simulink model "deltino"  (R2021b)
(part 9 of 10)

et152 = t27.*th33_dot.*(-1.6125e-2)+t28.*th41_dot.*(3.0./2.5e+2)-t29.*th42_dot.*1.6125e-2-t30.*th43_dot.*1.6125e-2-(t75.*th11_dot)./3.75e+2-(t76.*th12_dot)./1.5e+3-(t77.*th13_dot)./1.5e+3-(t78.*th21_dot)./3.75e+2-(t79.*th22_dot)./1.5e+3-(t80.*th23_dot)./1.5e+3-(t81.*th31_dot)./3.75e+2-(t82.*th32_dot)./1.5e+3-(t83.*th33_dot)./1.5e+3-(t84.*th41_dot)./3.75e+2-(t85.*th42_dot)./1.5e+3-(t86.*th43_dot)./1.5e+3-psi_dot.*t19.*t46.*(2.1e+1./1.0e+3)-psi_dot.*t20.*t46.*(2.1e+1./1.0e+3)-psi_dot.*t21.*t46.*(2.1e+1./1.0e+3);
et153 = psi_dot.*t22.*t46.*(2.1e+1./1.0e+3)+psi_dot.*t23.*t46.*(2.1e+1./1.0e+3)+psi_dot.*t24.*t46.*(2.1e+1./1.0e+3)+psi_dot.*t25.*t46.*(2.1e+1./1.0e+3)+psi_dot.*t26.*t46.*(2.1e+1./1.0e+3)+psi_dot.*t27.*t46.*(2.1e+1./1.0e+3)-psi_dot.*t28.*t46.*(2.1e+1./1.0e+3)-psi_dot.*t29.*t46.*(2.1e+1./1.0e+3)-psi_dot.*t30.*t46.*(2.1e+1./1.0e+3)+psi_dot.*t5.*t74.*6.75e-3+psi_dot.*t6.*t74.*6.75e-3+psi_dot.*t8.*t74.*6.75e-3+psi_dot.*t9.*t74.*6.75e-3+psi_dot.*t11.*t74.*6.75e-3+psi_dot.*t12.*t74.*6.75e-3+psi_dot.*t14.*t74.*6.75e-3+psi_dot.*t15.*t74.*6.75e-3-psi_dot.*t19.*t74.*(3.0./5.0e+2);
et154 = psi_dot.*t20.*t74.*(-3.0./5.0e+2)-psi_dot.*t21.*t74.*(3.0./5.0e+2)-psi_dot.*t22.*t74.*(3.0./5.0e+2)-psi_dot.*t23.*t74.*(3.0./5.0e+2)-psi_dot.*t24.*t74.*(3.0./5.0e+2)-psi_dot.*t25.*t74.*(3.0./5.0e+2)-psi_dot.*t26.*t74.*(3.0./5.0e+2)-psi_dot.*t27.*t74.*(3.0./5.0e+2)-psi_dot.*t28.*t74.*(3.0./5.0e+2)-psi_dot.*t29.*t74.*(3.0./5.0e+2)-psi_dot.*t30.*t74.*(3.0./5.0e+2)+(psi_dot.*t48.*t74)./3.75e+2+psi_dot.*t49.*t74.*4.666666666666667e-3+psi_dot.*t50.*t74.*4.666666666666667e-3+(psi_dot.*t51.*t74)./3.75e+2+psi_dot.*t52.*t74.*4.666666666666667e-3+psi_dot.*t53.*t74.*4.666666666666667e-3+(psi_dot.*t54.*t74)./3.75e+2+psi_dot.*t55.*t74.*4.666666666666667e-3+psi_dot.*t56.*t74.*4.666666666666667e-3;
et155 = (psi_dot.*t57.*t74)./3.75e+2+psi_dot.*t58.*t74.*4.666666666666667e-3+psi_dot.*t59.*t74.*4.666666666666667e-3+t4.*t46.*th11_dot.*(3.0./1.0e+3)+t5.*t46.*th12_dot.*(3.0./1.0e+3)+t6.*t46.*th13_dot.*(3.0./1.0e+3)+t7.*t46.*th21_dot.*(3.0./1.0e+3)+t8.*t46.*th22_dot.*(3.0./1.0e+3)+t9.*t46.*th23_dot.*(3.0./1.0e+3)+t20.*t46.*th12_dot.*3.375e-3+t21.*t46.*th13_dot.*3.375e-3+t10.*t46.*th31_dot.*(3.0./1.0e+3)-t4.*t74.*th11_dot.*1.05e-2+t11.*t46.*th32_dot.*(3.0./1.0e+3)-t5.*t74.*th12_dot.*1.05e-2+t12.*t46.*th33_dot.*(3.0./1.0e+3)+t23.*t46.*th22_dot.*3.375e-3-t6.*t74.*th13_dot.*1.05e-2+t24.*t46.*th23_dot.*3.375e-3;
et156 = t13.*t46.*th41_dot.*(3.0./1.0e+3)+t7.*t74.*th21_dot.*1.05e-2+t14.*t46.*th42_dot.*(3.0./1.0e+3)+t8.*t74.*th22_dot.*1.05e-2+t15.*t46.*th43_dot.*(3.0./1.0e+3)+t26.*t46.*th32_dot.*3.375e-3+t9.*t74.*th23_dot.*1.05e-2+t27.*t46.*th33_dot.*3.375e-3+t10.*t74.*th31_dot.*1.05e-2+t11.*t74.*th32_dot.*1.05e-2+t29.*t46.*th42_dot.*3.375e-3+t12.*t74.*th33_dot.*1.05e-2+t30.*t46.*th43_dot.*3.375e-3-t20.*t92.*th12_dot.*5.25e-3+t21.*t92.*th13_dot.*5.25e-3-t13.*t74.*th41_dot.*1.05e-2-t14.*t74.*th42_dot.*1.05e-2-t15.*t74.*th43_dot.*1.05e-2;
et157 = (t46.*t75.*th11_dot)./3.75e+2+t46.*t76.*th12_dot.*4.666666666666667e-3+t46.*t77.*th13_dot.*4.666666666666667e-3+t23.*t92.*th22_dot.*5.25e-3-t24.*t92.*th23_dot.*5.25e-3+(t46.*t78.*th21_dot)./3.75e+2+t46.*t79.*th22_dot.*4.666666666666667e-3+t46.*t80.*th23_dot.*4.666666666666667e-3+t26.*t92.*th32_dot.*5.25e-3-t27.*t92.*th33_dot.*5.25e-3+(t46.*t81.*th31_dot)./3.75e+2+t46.*t82.*th32_dot.*4.666666666666667e-3+t46.*t83.*th33_dot.*4.666666666666667e-3-t29.*t92.*th42_dot.*5.25e-3+t30.*t92.*th43_dot.*5.25e-3+(t46.*t84.*th41_dot)./3.75e+2+t46.*t85.*th42_dot.*4.666666666666667e-3+t46.*t86.*th43_dot.*4.666666666666667e-3-psi_dot.*t5.*t46.*t92.*(3.0./1.0e+3);
et158 = psi_dot.*t6.*t46.*t92.*(3.0./1.0e+3)-psi_dot.*t8.*t46.*t92.*(3.0./1.0e+3)+psi_dot.*t9.*t46.*t92.*(3.0./1.0e+3)-psi_dot.*t11.*t46.*t92.*(3.0./1.0e+3)+psi_dot.*t12.*t46.*t92.*(3.0./1.0e+3)-psi_dot.*t14.*t46.*t92.*(3.0./1.0e+3)+psi_dot.*t15.*t46.*t92.*(3.0./1.0e+3)-psi_dot.*t20.*t46.*t92.*4.5e-3+psi_dot.*t21.*t46.*t92.*4.5e-3-psi_dot.*t23.*t46.*t92.*4.5e-3+psi_dot.*t24.*t46.*t92.*4.5e-3-psi_dot.*t26.*t46.*t92.*4.5e-3+psi_dot.*t27.*t46.*t92.*4.5e-3-psi_dot.*t29.*t46.*t92.*4.5e-3+psi_dot.*t30.*t46.*t92.*4.5e-3+psi_dot.*t5.*t74.*t92.*1.05e-2;
et159 = psi_dot.*t6.*t74.*t92.*(-1.05e-2)-psi_dot.*t8.*t74.*t92.*1.05e-2+psi_dot.*t9.*t74.*t92.*1.05e-2-psi_dot.*t11.*t74.*t92.*1.05e-2+psi_dot.*t12.*t74.*t92.*1.05e-2+psi_dot.*t14.*t74.*t92.*1.05e-2-psi_dot.*t15.*t74.*t92.*1.05e-2-(psi_dot.*t46.*t76.*t92)./3.75e+2+(psi_dot.*t46.*t77.*t92)./3.75e+2-(psi_dot.*t46.*t79.*t92)./3.75e+2+(psi_dot.*t46.*t80.*t92)./3.75e+2-(psi_dot.*t46.*t82.*t92)./3.75e+2+(psi_dot.*t46.*t83.*t92)./3.75e+2-(psi_dot.*t46.*t85.*t92)./3.75e+2+(psi_dot.*t46.*t86.*t92)./3.75e+2+t20.*t46.*t92.*th12_dot.*5.25e-3-t21.*t46.*t92.*th13_dot.*5.25e-3;
et160 = t5.*t74.*t92.*th12_dot.*(-2.25e-3)-t23.*t46.*t92.*th22_dot.*5.25e-3+t6.*t74.*t92.*th13_dot.*2.25e-3+t24.*t46.*t92.*th23_dot.*5.25e-3-t8.*t74.*t92.*th22_dot.*2.25e-3-t26.*t46.*t92.*th32_dot.*5.25e-3+t9.*t74.*t92.*th23_dot.*2.25e-3+t20.*t74.*t92.*th12_dot.*1.5e-3+t27.*t46.*t92.*th33_dot.*5.25e-3-t21.*t74.*t92.*th13_dot.*1.5e-3-t11.*t74.*t92.*th32_dot.*2.25e-3+t29.*t46.*t92.*th42_dot.*5.25e-3+t12.*t74.*t92.*th33_dot.*2.25e-3+t23.*t74.*t92.*th22_dot.*1.5e-3-t30.*t46.*t92.*th43_dot.*5.25e-3-t24.*t74.*t92.*th23_dot.*1.5e-3;
et161 = t14.*t74.*t92.*th42_dot.*(-2.25e-3)+t15.*t74.*t92.*th43_dot.*2.25e-3+t26.*t74.*t92.*th32_dot.*1.5e-3-t27.*t74.*t92.*th33_dot.*1.5e-3-(t49.*t74.*t92.*th12_dot)./3.75e+2+(t50.*t74.*t92.*th13_dot)./3.75e+2+t29.*t74.*t92.*th42_dot.*1.5e-3-t30.*t74.*t92.*th43_dot.*1.5e-3-(t52.*t74.*t92.*th22_dot)./3.75e+2+(t53.*t74.*t92.*th23_dot)./3.75e+2-(t55.*t74.*t92.*th32_dot)./3.75e+2+(t56.*t74.*t92.*th33_dot)./3.75e+2-(t58.*t74.*t92.*th42_dot)./3.75e+2+(t59.*t74.*t92.*th43_dot)./3.75e+2;
et162 = -t138+t139+t140-t141+t142+t143-t144+t145+t146-t147+t148+t149+t189+t191+t193+t195+t197+t199+t201+t203+t205+t207+t209+t211-t329-t330-t331-t332-t333-t334-t335-t336-t337-t338-t339-t340+t341+t343+t345+t347+t351+t353-t355-t357+t406+t407+t408+t409+t410+t411+t412+t413-t470-t471-t472-t473+t503+t504+t506+t507+t509+t510+t512+t513-t567-t569-t571-t573-t575-t577-t579-t581+t598-t600-t601-t602-t603-t604-t605-t606-t607+t616+t617+t618+t619+t653;
et163 = t654+t655+t656-t683+t685+t687-t689+t691+t693-t695-t697+t699+t701-t703-t705+t707+t709+t711+t713-t715-t717-t719-t721+t769+t770+t771+t772+t773+t774+t775+t776+t777+t778+t779+t780+t829-t830-t831+t832-t833-t834+t835-t836-t837+t838-t839-t840-t889-t890-t891+t892+t893+t894+t895+t896+t897-t898-t899-t900+t901+t902+t903+t904+t905+t906+t907+t908+t934+t951+t952+t953+t954+t955+t956+t957+t958-t1275-t1276-t1277+t1278+t1279+t1280+t1281+t1282+t1283-t1284-t1285-t1286-t1340-t1341-t1342-t1343-t1344;
et164 = -t1345-t1346-t1347+t1444-t1445+t1446-t1447+t1449+t1451-t1458+t1464-t1465-t1468+t1469-t1472+t1473+t1474-t1475-t1549+t1550-t1551+t1552-t1553+t1554-t1555+t1556+t1571+t1573+t1575+t1577+t1646+t1647+t1648+t1649-t1675+t1676-t1677+t1678+t1679-t1680-t1681+t1682-t1683+t1684-t1685+t1686-t1687+t1688+t1689-t1690-t1751+t1752-t1753+t1754-t1755+t1756-t1757+t1758-t1808+t1809-t1810+t1811-t1812+t1813-t1814+t1815+t1849-t1850+t1851-t1852+t1853-t1854+t1855-t1856+t1878+t1879+t1881+t1884-t1933+t1934-t1935+t1936-t1937+t1938-t1939+t1940;
et165 = -t2002+t2003-t2004+t2005-t2006+t2007-t2008+t2009-psi_dot.*t3.*t4.*(3.0./5.0e+2)+psi_dot.*t3.*t5.*(3.0./1.0e+3)+psi_dot.*t3.*t6.*(3.0./1.0e+3)-psi_dot.*t3.*t7.*(3.0./5.0e+2)+psi_dot.*t3.*t8.*(3.0./1.0e+3)+psi_dot.*t3.*t9.*(3.0./1.0e+3)-psi_dot.*t3.*t10.*(3.0./5.0e+2)+psi_dot.*t3.*t11.*(3.0./1.0e+3)+psi_dot.*t3.*t12.*(3.0./1.0e+3)-psi_dot.*t3.*t13.*(3.0./5.0e+2)+psi_dot.*t3.*t14.*(3.0./1.0e+3)+psi_dot.*t3.*t15.*(3.0./1.0e+3)-psi_dot.*t3.*t19.*(3.0./1.0e+2)+psi_dot.*t4.*t18.*(2.1e+1./1.0e+3)-psi_dot.*t3.*t20.*1.65e-2-psi_dot.*t5.*t18.*1.05e-2-psi_dot.*t3.*t21.*1.65e-2;
et166 = psi_dot.*t6.*t18.*(-1.05e-2)-psi_dot.*t3.*t22.*(3.0./1.0e+2)-psi_dot.*t7.*t18.*(2.1e+1./1.0e+3)-psi_dot.*t3.*t23.*1.65e-2+psi_dot.*t8.*t18.*1.05e-2-psi_dot.*t3.*t24.*1.65e-2+psi_dot.*t9.*t18.*1.05e-2+psi_dot.*t3.*t25.*(3.0./2.5e+2)-psi_dot.*t10.*t18.*(2.1e+1./1.0e+3)+psi_dot.*t3.*t26.*2.55e-2+psi_dot.*t11.*t18.*1.05e-2+psi_dot.*t3.*t27.*2.55e-2+psi_dot.*t12.*t18.*1.05e-2+psi_dot.*t3.*t28.*(3.0./2.5e+2)+psi_dot.*t13.*t18.*(2.1e+1./1.0e+3)+psi_dot.*t3.*t29.*2.55e-2-psi_dot.*t14.*t18.*1.05e-2+psi_dot.*t3.*t30.*2.55e-2;
et167 = psi_dot.*t15.*t18.*(-1.05e-2)-psi_dot.*t3.*t75.*(2.0./3.75e+2)+(psi_dot.*t3.*t76)./3.75e+2+(psi_dot.*t3.*t77)./3.75e+2-psi_dot.*t3.*t78.*(2.0./3.75e+2)+(psi_dot.*t3.*t79)./3.75e+2+(psi_dot.*t3.*t80)./3.75e+2-psi_dot.*t3.*t81.*(2.0./3.75e+2)+(psi_dot.*t3.*t82)./3.75e+2+(psi_dot.*t3.*t83)./3.75e+2-psi_dot.*t3.*t84.*(2.0./3.75e+2)+(psi_dot.*t3.*t85)./3.75e+2+(psi_dot.*t3.*t86)./3.75e+2+t18.*t92.*t125+t18.*t92.*t128-t4.*t18.*th11_dot.*(3.0./1.0e+2)-t5.*t18.*th12_dot.*1.65e-2-t6.*t18.*th13_dot.*1.65e-2-t7.*t18.*th21_dot.*(3.0./1.0e+2)-t8.*t18.*th22_dot.*1.65e-2-t9.*t18.*th23_dot.*1.65e-2;
et168 = t10.*t18.*th31_dot.*(3.0./2.5e+2)+t11.*t18.*th32_dot.*2.55e-2+t12.*t18.*th33_dot.*2.55e-2+t13.*t18.*th41_dot.*(3.0./2.5e+2)+t14.*t18.*th42_dot.*2.55e-2+t15.*t18.*th43_dot.*2.55e-2-phi_dot.*t5.*t16.*t46.*6.75e-3-phi_dot.*t6.*t16.*t46.*6.75e-3-phi_dot.*t8.*t16.*t46.*6.75e-3-phi_dot.*t9.*t16.*t46.*6.75e-3-phi_dot.*t11.*t16.*t46.*6.75e-3-phi_dot.*t12.*t16.*t46.*6.75e-3-phi_dot.*t14.*t16.*t46.*6.75e-3-phi_dot.*t15.*t16.*t46.*6.75e-3-(phi_dot.*t16.*t46.*t48)./3.75e+2-(phi_dot.*t16.*t46.*t51)./3.75e+2-(phi_dot.*t16.*t46.*t54)./3.75e+2;
et169 = phi_dot.*t16.*t46.*t57.*(-1.0./3.75e+2)-psi_dot.*t6.*t18.*t92.*(3.0./5.0e+2)-psi_dot.*t9.*t18.*t92.*(3.0./5.0e+2)-psi_dot.*t11.*t18.*t92.*(3.0./2.0e+2)+psi_dot.*t12.*t18.*t92.*(3.0./2.0e+2)-psi_dot.*t14.*t18.*t92.*(3.0./2.0e+2)+psi_dot.*t15.*t18.*t92.*(3.0./2.0e+2)-(psi_dot.*t18.*t49.*t92)./7.5e+2+(psi_dot.*t18.*t50.*t92)./7.5e+2-(psi_dot.*t18.*t52.*t92)./7.5e+2+(psi_dot.*t18.*t53.*t92)./7.5e+2-(psi_dot.*t18.*t55.*t92)./7.5e+2+(psi_dot.*t18.*t56.*t92)./7.5e+2-(psi_dot.*t18.*t58.*t92)./7.5e+2+(psi_dot.*t18.*t59.*t92)./7.5e+2+t3.*t20.*t92.*th12_dot.*8.25e-3-t3.*t21.*t92.*th13_dot.*8.25e-3;
et170 = t3.*t23.*t92.*th22_dot.*8.25e-3-t3.*t24.*t92.*th23_dot.*8.25e-3-t3.*t26.*t92.*th32_dot.*1.275e-2+t3.*t27.*t92.*th33_dot.*1.275e-2-t3.*t29.*t92.*th42_dot.*1.275e-2+t3.*t30.*t92.*th43_dot.*1.275e-2-phi_dot.*t5.*t18.*t31.*t92.*(3.0./5.0e+2)-phi_dot.*t8.*t18.*t31.*t92.*(3.0./5.0e+2)-phi_dot.*t5.*t16.*t46.*t92.*1.05e-2-phi_dot.*t9.*t16.*t46.*t92.*1.05e-2-phi_dot.*t12.*t16.*t46.*t92.*1.05e-2-phi_dot.*t14.*t16.*t46.*t92.*1.05e-2;
et171 = t304+t305+t306+t307+t308+t309+t310+t311+t312+t313+t314+t315+t462+t463+t464+t465+t466+t467+t468+t469+t586+t587+t588+t589+t590+t591+t592+t593+t594+t595+t596+t597-t667-t668+t669+t670+t753+t756+t759+t762-t817-t818-t819-t820-t821-t822-t824-t825-t827-t828+t877+t878+t879-t880-t881-t882-t883-t884-t885+t886+t887+t888+t961+t963+t965+t967+t969+t971+t973+t975+t976+t977+t978-t979-t980-t981-t982-t983-t984+t985+t986+t987+t1002+t1003+t1004+t1005+t1006+t1007+t1008+t1009+t1054+t1055+t1056+t1057+t1058+t1059+t1060+t1061+t1062+t1063+t1064+t1065-t1106+t1107+t1108-t1109+t1110+t1111-t1112+t1113+t1114-t1115+t1116+t1117+t1119+t1120;
et172 = t1122+t1123-t1124-t1125-t1128-t1129+t1132+t1133-t1162-t1163-t1166-t1167+t1170+t1171+t1172+t1173-t1183-t1184-t1185-t1186-t1187-t1188-t1190-t1191-t1193-t1194+t1247+t1248+t1249+t1250+t1251+t1252+t1253+t1254+t1307+t1332+t1335+t1337+t1338-t1360-t1361-t1362+t1363+t1364+t1365+t1366+t1367+t1368-t1369-t1370-t1371+t1512+t1513+t1514+t1515+t1541-t1542+t1543-t1544+t1545-t1546+t1547-t1548+t1590+t1591+t1592+t1593+t1594+t1595+t1596+t1597+t1598+t1608+t1609+t1610+t1611+t1612+t1613+t1614+t1615+t1616+t1617+t1618+t1619+t1637+t1639+t1641+t1643+t1659-t1660+t1661-t1662+t1665-t1666+t1669-t1670+t1711-t1712+t1713;
et173 = -t1714+t1716+t1718+t1719+t1721+t1723+t1725+t1760+t1762+t1764+t1766+t1865+t1866+t1867+t1868+t1869-t1870+t1871-t1872+t1873-t1874+t1875-t1876+t1909+t1912+t1914+t1915+t1971+t1973+t1975+t1977+t1994-t1995+t1996-t1997+t1998-t1999+t2000-t2001+t2034-t2035+t2036-t2037+t2038-t2039+t2040-t2041-t2108+t2109-t2110+t2111-t2112+t2113-t2114+t2115-t2124+t2125-t2126+t2127-t2128+t2129-t2130+t2131+t2150+t2153+t2155+t2156-t16.*zeta_dot.*6.720125e-1+t3.*t31.*t153+t3.*t31.*t154-t3.*t16.*th11_dot.*(4.0./3.75e+2)+t3.*t16.*th12_dot.*(2.0./3.75e+2)+t3.*t16.*th13_dot.*(2.0./3.75e+2)-t3.*t16.*th21_dot.*(4.0./3.75e+2);
et174 = t3.*t16.*th22_dot.*(2.0./3.75e+2)+t3.*t16.*th23_dot.*(2.0./3.75e+2)-t3.*t16.*th31_dot.*(4.0./3.75e+2)+t3.*t16.*th32_dot.*(2.0./3.75e+2)+t3.*t16.*th33_dot.*(2.0./3.75e+2)-t3.*t16.*th41_dot.*(4.0./3.75e+2)+t3.*t16.*th42_dot.*(2.0./3.75e+2)+t3.*t16.*th43_dot.*(2.0./3.75e+2)-t5.*t16.*zeta_dot.*1.35e-2-t6.*t16.*zeta_dot.*1.35e-2-t8.*t16.*zeta_dot.*1.35e-2-t9.*t16.*zeta_dot.*1.35e-2-t11.*t16.*zeta_dot.*1.35e-2-t12.*t16.*zeta_dot.*1.35e-2-t14.*t16.*zeta_dot.*1.35e-2-t15.*t16.*zeta_dot.*1.35e-2-(t16.*t61.*zeta_dot)./1.25e+2-(t16.*t62.*zeta_dot)./1.25e+2-(t16.*t64.*zeta_dot)./1.25e+2;
et175 = t16.*t65.*zeta_dot.*(-1.0./1.25e+2)-(t16.*t67.*zeta_dot)./1.25e+2-(t16.*t68.*zeta_dot)./1.25e+2-(t16.*t70.*zeta_dot)./1.25e+2-(t16.*t71.*zeta_dot)./1.25e+2-t3.*t16.*t19.*th11_dot.*(3.0./5.0e+2)+t3.*t16.*t20.*th12_dot.*(3.0./1.0e+3)+t3.*t16.*t21.*th13_dot.*(3.0./1.0e+3)-t3.*t16.*t22.*th21_dot.*(3.0./5.0e+2)+t3.*t16.*t23.*th22_dot.*(3.0./1.0e+3)+t16.*t18.*t19.*th11_dot.*(2.1e+1./1.0e+3)+t3.*t16.*t24.*th23_dot.*(3.0./1.0e+3)-t16.*t18.*t20.*th12_dot.*1.05e-2-t16.*t18.*t21.*th13_dot.*1.05e-2-t3.*t16.*t25.*th31_dot.*(3.0./5.0e+2)+t3.*t16.*t26.*th32_dot.*(3.0./1.0e+3)-t16.*t18.*t22.*th21_dot.*(2.1e+1./1.0e+3)+t3.*t16.*t27.*th33_dot.*(3.0./1.0e+3);
et176 = t16.*t18.*t23.*th22_dot.*1.05e-2+t16.*t18.*t24.*th23_dot.*1.05e-2-t3.*t16.*t28.*th41_dot.*(3.0./5.0e+2)+t3.*t16.*t29.*th42_dot.*(3.0./1.0e+3)-t16.*t18.*t25.*th31_dot.*(2.1e+1./1.0e+3)+t3.*t16.*t30.*th43_dot.*(3.0./1.0e+3)+t16.*t18.*t26.*th32_dot.*1.05e-2+t16.*t18.*t27.*th33_dot.*1.05e-2+t16.*t18.*t28.*th41_dot.*(2.1e+1./1.0e+3)-t16.*t18.*t29.*th42_dot.*1.05e-2-t16.*t18.*t30.*th43_dot.*1.05e-2-t3.*t4.*t31.*zeta_dot.*(3.0./5.0e+2)+t3.*t5.*t31.*zeta_dot.*(3.0./1.0e+3)+t3.*t6.*t31.*zeta_dot.*(3.0./1.0e+3)-t3.*t7.*t31.*zeta_dot.*(3.0./5.0e+2)+t3.*t8.*t31.*zeta_dot.*(3.0./1.0e+3)+t3.*t9.*t31.*zeta_dot.*(3.0./1.0e+3);
et177 = t3.*t10.*t31.*zeta_dot.*(-3.0./5.0e+2)+t3.*t11.*t31.*zeta_dot.*(3.0./1.0e+3)+t3.*t12.*t31.*zeta_dot.*(3.0./1.0e+3)-t3.*t13.*t31.*zeta_dot.*(3.0./5.0e+2)+t3.*t14.*t31.*zeta_dot.*(3.0./1.0e+3)+t3.*t15.*t31.*zeta_dot.*(3.0./1.0e+3)-t3.*t19.*t31.*zeta_dot.*(3.0./1.0e+2)+t4.*t18.*t31.*zeta_dot.*(2.1e+1./1.0e+3)-t3.*t20.*t31.*zeta_dot.*1.65e-2-t5.*t18.*t31.*zeta_dot.*1.05e-2-t3.*t21.*t31.*zeta_dot.*1.65e-2-t6.*t18.*t31.*zeta_dot.*1.05e-2-t3.*t22.*t31.*zeta_dot.*(3.0./1.0e+2)-t7.*t18.*t31.*zeta_dot.*(2.1e+1./1.0e+3)-t3.*t23.*t31.*zeta_dot.*1.65e-2+t8.*t18.*t31.*zeta_dot.*1.05e-2;
et178 = t3.*t24.*t31.*zeta_dot.*(-1.65e-2)+t9.*t18.*t31.*zeta_dot.*1.05e-2-t10.*t18.*t31.*zeta_dot.*(2.1e+1./1.0e+3)+t3.*t26.*t31.*zeta_dot.*2.55e-2+t11.*t18.*t31.*zeta_dot.*1.05e-2+t3.*t27.*t31.*zeta_dot.*2.55e-2+t12.*t18.*t31.*zeta_dot.*1.05e-2+t13.*t18.*t31.*zeta_dot.*(2.1e+1./1.0e+3)+t3.*t29.*t31.*zeta_dot.*2.55e-2-t14.*t18.*t31.*zeta_dot.*1.05e-2+t3.*t30.*t31.*zeta_dot.*2.55e-2-t15.*t18.*t31.*zeta_dot.*1.05e-2-t16.*t25.*t47.*zeta_dot.*(3.0./2.5e+2)-t16.*t28.*t47.*zeta_dot.*(3.0./2.5e+2)-t5.*t16.*t92.*zeta_dot.*(2.1e+1./1.0e+3)+t6.*t16.*t92.*zeta_dot.*(2.1e+1./1.0e+3);
et179 = t8.*t16.*t92.*zeta_dot.*(2.1e+1./1.0e+3)-t9.*t16.*t92.*zeta_dot.*(2.1e+1./1.0e+3)+t11.*t16.*t92.*zeta_dot.*(2.1e+1./1.0e+3)-t12.*t16.*t92.*zeta_dot.*(2.1e+1./1.0e+3)-t14.*t16.*t92.*zeta_dot.*(2.1e+1./1.0e+3)+t15.*t16.*t92.*zeta_dot.*(2.1e+1./1.0e+3)-phi_dot.*t3.*t4.*t16.*t31.*(2.1e+1./1.0e+3)-phi_dot.*t3.*t13.*t16.*t31.*(2.1e+1./1.0e+3)-phi_dot.*t4.*t16.*t18.*t31.*(3.0./5.0e+2)-phi_dot.*t7.*t16.*t18.*t31.*(3.0./5.0e+2)-phi_dot.*t10.*t16.*t18.*t31.*(3.0./5.0e+2)-phi_dot.*t13.*t16.*t18.*t31.*(3.0./5.0e+2)-phi_dot.*t3.*t18.*t25.*t73.*(3.0./2.5e+2)-phi_dot.*t3.*t18.*t28.*t73.*(3.0./2.5e+2)-phi_dot.*t6.*t21.*t73.*t92.*(2.0./3.75e+2)-phi_dot.*t9.*t24.*t73.*t92.*(2.0./3.75e+2);
et180 = phi_dot.*t12.*t27.*t73.*t92.*(-2.0./3.75e+2)-phi_dot.*t15.*t30.*t73.*t92.*(2.0./3.75e+2)-phi_dot.*t5.*t47.*t73.*t92.*(3.0./5.0e+2)-phi_dot.*t8.*t47.*t73.*t92.*(3.0./5.0e+2)-phi_dot.*t11.*t47.*t73.*t92.*(3.0./5.0e+2)-phi_dot.*t14.*t47.*t73.*t92.*(3.0./5.0e+2)-t16.*t18.*t20.*t92.*th12_dot.*2.25e-3+t16.*t18.*t21.*t92.*th13_dot.*2.25e-3-t16.*t18.*t23.*t92.*th22_dot.*2.25e-3+t16.*t18.*t24.*t92.*th23_dot.*2.25e-3-t16.*t18.*t26.*t92.*th32_dot.*2.25e-3+t16.*t18.*t27.*t92.*th33_dot.*2.25e-3-t16.*t18.*t29.*t92.*th42_dot.*2.25e-3+t16.*t18.*t30.*t92.*th43_dot.*2.25e-3-t3.*t4.*t19.*t31.*zeta_dot.*(4.0./3.75e+2);
et181 = t3.*t5.*t20.*t31.*zeta_dot.*(2.0./3.75e+2)+t3.*t6.*t21.*t31.*zeta_dot.*(2.0./3.75e+2)-t3.*t7.*t22.*t31.*zeta_dot.*(4.0./3.75e+2)+t3.*t8.*t23.*t31.*zeta_dot.*(2.0./3.75e+2)+t3.*t9.*t24.*t31.*zeta_dot.*(2.0./3.75e+2)-t3.*t10.*t25.*t31.*zeta_dot.*(4.0./3.75e+2)+t3.*t11.*t26.*t31.*zeta_dot.*(2.0./3.75e+2)+t3.*t12.*t27.*t31.*zeta_dot.*(2.0./3.75e+2)-t3.*t13.*t28.*t31.*zeta_dot.*(4.0./3.75e+2)+t3.*t14.*t29.*t31.*zeta_dot.*(2.0./3.75e+2)+t3.*t15.*t30.*t31.*zeta_dot.*(2.0./3.75e+2)+t5.*t18.*t31.*t92.*zeta_dot.*(3.0./5.0e+2)-t6.*t18.*t31.*t92.*zeta_dot.*(3.0./5.0e+2)+t8.*t18.*t31.*t92.*zeta_dot.*(3.0./5.0e+2)-t9.*t18.*t31.*t92.*zeta_dot.*(3.0./5.0e+2)-t11.*t18.*t31.*t92.*zeta_dot.*(3.0./2.0e+2)+t12.*t18.*t31.*t92.*zeta_dot.*(3.0./2.0e+2);
et182 = t14.*t18.*t31.*t92.*zeta_dot.*(-3.0./2.0e+2)+t15.*t18.*t31.*t92.*zeta_dot.*(3.0./2.0e+2)-t6.*t16.*t47.*t92.*zeta_dot.*(2.1e+1./1.0e+3)-t8.*t16.*t47.*t92.*zeta_dot.*(2.1e+1./1.0e+3)-t11.*t16.*t47.*t92.*zeta_dot.*(2.1e+1./1.0e+3)-t15.*t16.*t47.*t92.*zeta_dot.*(2.1e+1./1.0e+3)-(t18.*t31.*t61.*t92.*zeta_dot)./3.75e+2+(t18.*t31.*t62.*t92.*zeta_dot)./3.75e+2-(t18.*t31.*t64.*t92.*zeta_dot)./3.75e+2+(t18.*t31.*t65.*t92.*zeta_dot)./3.75e+2-(t18.*t31.*t67.*t92.*zeta_dot)./3.75e+2+(t18.*t31.*t68.*t92.*zeta_dot)./3.75e+2-(t18.*t31.*t70.*t92.*zeta_dot)./3.75e+2+(t18.*t31.*t71.*t92.*zeta_dot)./3.75e+2-phi_dot.*t3.*t5.*t16.*t31.*t92.*(3.0./5.0e+2)-phi_dot.*t3.*t8.*t16.*t31.*t92.*(3.0./5.0e+2);
et183 = phi_dot.*t3.*t6.*t18.*t73.*t92.*(-2.1e+1./1.0e+3)-phi_dot.*t3.*t8.*t18.*t73.*t92.*(2.1e+1./1.0e+3)-phi_dot.*t3.*t11.*t18.*t73.*t92.*(2.1e+1./1.0e+3)-phi_dot.*t3.*t15.*t18.*t73.*t92.*(2.1e+1./1.0e+3)-t3.*t6.*t16.*t18.*t92.*zeta_dot.*(3.0./5.0e+2)-t3.*t9.*t16.*t18.*t92.*zeta_dot.*(3.0./5.0e+2)-t3.*t12.*t16.*t18.*t92.*zeta_dot.*(3.0./5.0e+2)-t3.*t15.*t16.*t18.*t92.*zeta_dot.*(3.0./5.0e+2);
et184 = t138-t139-t140+t141-t142-t143+t144-t145-t146+t147-t148-t149-t189-t191-t193-t195-t197-t199-t201-t203-t205-t207-t209-t211+t329+t330+t331+t332+t333+t334+t335+t336+t337+t338+t339+t340-t351-t353+t355+t357-t406-t407-t408-t409-t410-t411-t412-t413+t470+t471+t472+t473+t503+t504+t506+t507+t509+t510+t512+t513+t567+t569+t571+t573+t575+t577+t579+t581-t598+t600+t601+t602+t603+t604+t605+t606+t607+t616+t617+t618+t619-t653-t654-t655-t656+t683-t685-t687+t689;
et185 = -t691-t693+t695+t697-t699-t701+t703+t705-t707-t709-t711-t713+t715+t717+t719+t721+t830+t831+t833+t834+t836+t837+t839+t840+t889+t890+t891-t892-t893-t894-t895-t896-t897+t898+t899+t900-t901-t902-t903-t904-t905-t906-t907-t908-t934-t951-t952-t953-t954-t955-t956-t957-t958+t1034+t1035+t1036+t1037+t1195+t1196+t1197+t1198+t1199+t1200+t1201+t1202+t1275+t1276+t1277-t1278-t1279-t1280-t1281-t1282-t1283+t1284+t1285+t1286+t1340+t1341+t1342+t1343+t1344+t1345+t1346+t1347-t1444;
et186 = t1445-t1446+t1447+t1448+t1450+t1458-t1464+t1465+t1468-t1469+t1472-t1473-t1474+t1475+t1549-t1550+t1551-t1552+t1553-t1554+t1555-t1556+t1571+t1573+t1575+t1577+t1646+t1647+t1648+t1649+t1675-t1676+t1677-t1678-t1679+t1680+t1681-t1682+t1683-t1684+t1685-t1686+t1687-t1688-t1689+t1690+t1751-t1752+t1753-t1754+t1755-t1756+t1757-t1758+t1808-t1809+t1810-t1811+t1812-t1813+t1814-t1815-t1849+t1850-t1851+t1852-t1853+t1854-t1855+t1856+t1877+t1880+t1882+t1883+t1933-t1934+t1935-t1936+t1937-t1938+t1939-t1940+t2002-t2003+t2004-t2005+t2006-t2007+t2008;
et187 = -t2009+t3.*t19.*th11_dot.*(2.1e+1./1.0e+3)-t3.*t20.*th12_dot.*1.05e-2-t3.*t21.*th13_dot.*1.05e-2-t3.*t22.*th21_dot.*(2.1e+1./1.0e+3)+t3.*t23.*th22_dot.*1.05e-2+t18.*t19.*th11_dot.*(3.0./5.0e+2)+t3.*t24.*th23_dot.*1.05e-2-t18.*t20.*th12_dot.*(3.0./1.0e+3)-t18.*t21.*th13_dot.*(3.0./1.0e+3)-t3.*t25.*th31_dot.*(2.1e+1./1.0e+3)+t3.*t26.*th32_dot.*1.05e-2+t18.*t22.*th21_dot.*(3.0./5.0e+2)+t3.*t27.*th33_dot.*1.05e-2-t18.*t23.*th22_dot.*(3.0./1.0e+3)-t18.*t24.*th23_dot.*(3.0./1.0e+3)+t3.*t28.*th41_dot.*(2.1e+1./1.0e+3)-t3.*t29.*th42_dot.*1.05e-2;
et188 = t18.*t25.*th31_dot.*(3.0./5.0e+2)-t3.*t30.*th43_dot.*1.05e-2-t18.*t26.*th32_dot.*(3.0./1.0e+3)-t18.*t27.*th33_dot.*(3.0./1.0e+3)+t18.*t28.*th41_dot.*(3.0./5.0e+2)-t18.*t29.*th42_dot.*(3.0./1.0e+3)-t18.*t30.*th43_dot.*(3.0./1.0e+3)-phi_dot.*t3.*t4.*t31.*(3.0./5.0e+2)-phi_dot.*t3.*t7.*t31.*(3.0./5.0e+2)-phi_dot.*t3.*t10.*t31.*(3.0./5.0e+2)-phi_dot.*t3.*t13.*t31.*(3.0./5.0e+2)-phi_dot.*t16.*t19.*t46.*(3.0./5.0e+2)-phi_dot.*t16.*t20.*t46.*(3.0./5.0e+2)-phi_dot.*t16.*t21.*t46.*(3.0./5.0e+2)-phi_dot.*t16.*t22.*t46.*(3.0./5.0e+2)-phi_dot.*t16.*t23.*t46.*(3.0./5.0e+2)-phi_dot.*t16.*t24.*t46.*(3.0./5.0e+2)-phi_dot.*t16.*t25.*t46.*(3.0./5.0e+2);
et189 = phi_dot.*t16.*t26.*t46.*(-3.0./5.0e+2)-phi_dot.*t16.*t27.*t46.*(3.0./5.0e+2)-phi_dot.*t16.*t28.*t46.*(3.0./5.0e+2)-phi_dot.*t16.*t29.*t46.*(3.0./5.0e+2)-phi_dot.*t16.*t30.*t46.*(3.0./5.0e+2)-phi_dot.*t3.*t31.*t75.*(2.0./3.75e+2)-phi_dot.*t3.*t31.*t78.*(2.0./3.75e+2)-phi_dot.*t3.*t31.*t81.*(2.0./3.75e+2)-phi_dot.*t3.*t31.*t84.*(2.0./3.75e+2)-t3.*t20.*t92.*th12_dot.*2.25e-3+t3.*t21.*t92.*th13_dot.*2.25e-3-t3.*t23.*t92.*th22_dot.*2.25e-3+t3.*t24.*t92.*th23_dot.*2.25e-3-t3.*t26.*t92.*th32_dot.*2.25e-3+t3.*t27.*t92.*th33_dot.*2.25e-3-t3.*t29.*t92.*th42_dot.*2.25e-3+t3.*t30.*t92.*th43_dot.*2.25e-3;
et190 = phi_dot.*t6.*t18.*t31.*t92.*(-3.0./5.0e+2)-phi_dot.*t9.*t18.*t31.*t92.*(3.0./5.0e+2)-phi_dot.*t6.*t16.*t46.*t92.*1.05e-2-phi_dot.*t8.*t16.*t46.*t92.*1.05e-2-phi_dot.*t11.*t16.*t46.*t92.*1.05e-2-phi_dot.*t15.*t16.*t46.*t92.*1.05e-2;
et191 = t4.*th11_dot.*(3.0./5.0e+2)+t5.*th12_dot.*(3.0./5.0e+2)+t6.*th13_dot.*(3.0./5.0e+2)+t7.*th21_dot.*(3.0./5.0e+2)+t8.*th22_dot.*(3.0./5.0e+2)+t9.*th23_dot.*(3.0./5.0e+2)-t20.*th12_dot.*6.75e-3-t21.*th13_dot.*6.75e-3+t10.*th31_dot.*(3.0./5.0e+2)+t11.*th32_dot.*(3.0./5.0e+2)+t12.*th33_dot.*(3.0./5.0e+2)-t23.*th22_dot.*6.75e-3-t24.*th23_dot.*6.75e-3+t13.*th41_dot.*(3.0./5.0e+2)+t14.*th42_dot.*(3.0./5.0e+2)+t15.*th43_dot.*(3.0./5.0e+2)-t26.*th32_dot.*6.75e-3-t27.*th33_dot.*6.75e-3-t29.*th42_dot.*6.75e-3-t30.*th43_dot.*6.75e-3+t75.*th11_dot.*(2.0./3.75e+2);
et192 = (t76.*th12_dot)./7.5e+2+(t77.*th13_dot)./7.5e+2+t78.*th21_dot.*(2.0./3.75e+2)+(t79.*th22_dot)./7.5e+2+(t80.*th23_dot)./7.5e+2+t81.*th31_dot.*(2.0./3.75e+2)+(t82.*th32_dot)./7.5e+2+(t83.*th33_dot)./7.5e+2+t84.*th41_dot.*(2.0./3.75e+2)+(t85.*th42_dot)./7.5e+2+(t86.*th43_dot)./7.5e+2-t20.*t92.*th12_dot.*1.05e-2+t21.*t92.*th13_dot.*1.05e-2+t23.*t92.*th22_dot.*1.05e-2-t24.*t92.*th23_dot.*1.05e-2+t26.*t92.*th32_dot.*1.05e-2-t27.*t92.*th33_dot.*1.05e-2-t29.*t92.*th42_dot.*1.05e-2+t30.*t92.*th43_dot.*1.05e-2;
et193 = -t113+t214+t266-t286+t303+t349+t369-t524-t638+t741-t794+t865+t917+t960+t1039-t1091+t1126-t1146-t1236+t1401+t1402+t1501+t1532-t1579+t1620+t1743+t1779+t1841-t1917-t1986+t2050-t2100+t2132-t2158-psi_dot.*t20.*t31.*6.75e-3+t5.*t16.*zeta_dot.*(2.1e+1./1.0e+3)-phi_dot.*t20.*t73.*t92.*1.05e-2-psi_dot.*t3.*t16.*t20.*(3.0./1.0e+3)+psi_dot.*t16.*t18.*t20.*1.05e-2-psi_dot.*t20.*t31.*t92.*1.05e-2-t5.*t18.*t31.*zeta_dot.*1.65e-2+t5.*t16.*t92.*zeta_dot.*4.5e-3-phi_dot.*t16.*t18.*t20.*t31.*1.05e-2-phi_dot.*t3.*t16.*t31.*t61.*(4.0./3.75e+2);
et194 = psi_dot.*t16.*t18.*t20.*t92.*2.25e-3+t3.*t20.*t31.*t92.*zeta_dot.*8.25e-3-t3.*t16.*t18.*t20.*t92.*zeta_dot.*1.05e-2-(t3.*t5.*t20.*t31.*t92.*zeta_dot)./3.75e+2-phi_dot.*t5.*t16.*t18.*t20.*t31.*t92.*(2.0./3.75e+2);
et195 = -t114+t216+t267-t287+t303+t349+t371-t525-t639+t743-t795+t867-t918+t962+t1040-t1092+t1127-t1147-t1237+t1325+t1502+t1533+t1569-t1580+t1664-t1744+t1768+t1807-t1842+t1918+t1987+t2019+t2043-t2051+t2101+t2159-psi_dot.*t21.*t31.*6.75e-3+t6.*t16.*zeta_dot.*(2.1e+1./1.0e+3)-psi_dot.*t3.*t16.*t21.*(3.0./1.0e+3)+psi_dot.*t16.*t18.*t21.*1.05e-2-t6.*t18.*t31.*zeta_dot.*1.65e-2-t6.*t16.*t92.*zeta_dot.*4.5e-3-t16.*t62.*t92.*zeta_dot.*(2.0./3.75e+2)-phi_dot.*t16.*t18.*t21.*t31.*1.05e-2-phi_dot.*t3.*t16.*t31.*t62.*(4.0./3.75e+2)-phi_dot.*t21.*t47.*t73.*t92.*1.05e-2;
et196 = psi_dot.*t16.*t18.*t21.*t92.*(-2.25e-3)-t3.*t21.*t31.*t92.*zeta_dot.*8.25e-3-phi_dot.*t16.*t18.*t21.*t31.*t92.*(3.0./5.0e+2);
et197 = -t116+t220+t268-t288+t303+t349+t372-t526-t641+t744-t797+t868-t919+t964+t1042-t1094+t1130-t1148+t1160+t1239+t1326+t1401+t1404+t1504+t1534+t1582+t1620+t1667+t1745+t1781+t1843-t1919-t1988+t2044+t2052-t2102-t2160-psi_dot.*t23.*t31.*6.75e-3-t8.*t16.*zeta_dot.*(2.1e+1./1.0e+3)-psi_dot.*t3.*t16.*t23.*(3.0./1.0e+3)-psi_dot.*t16.*t18.*t23.*1.05e-2-t8.*t18.*t31.*zeta_dot.*1.65e-2+t8.*t16.*t92.*zeta_dot.*4.5e-3-phi_dot.*t3.*t16.*t31.*t64.*(4.0./3.75e+2)-phi_dot.*t23.*t47.*t73.*t92.*1.05e-2+psi_dot.*t16.*t18.*t23.*t92.*2.25e-3+t3.*t23.*t31.*t92.*zeta_dot.*8.25e-3;
et198 = t3.*t8.*t23.*t31.*t92.*zeta_dot.*(-1.0./3.75e+2)-phi_dot.*t8.*t16.*t18.*t23.*t31.*t92.*(2.0./3.75e+2);
et199 = -t117+t222+t269-t289+t303+t349+t374-t527-t642+t746-t798+t870+t920+t966+t1043-t1095+t1131-t1149+t1161+t1240+t1505+t1535+t1569+t1583-t1746+t1770+t1807-t1844+t1920+t1989+t2021-t2053+t2103+t2135+t2161-psi_dot.*t24.*t31.*6.75e-3-t9.*t16.*zeta_dot.*(2.1e+1./1.0e+3)-phi_dot.*t24.*t73.*t92.*1.05e-2-psi_dot.*t3.*t16.*t24.*(3.0./1.0e+3)-psi_dot.*t16.*t18.*t24.*1.05e-2-psi_dot.*t24.*t31.*t92.*1.05e-2-t9.*t18.*t31.*zeta_dot.*1.65e-2-t9.*t16.*t92.*zeta_dot.*4.5e-3-t16.*t65.*t92.*zeta_dot.*(2.0./3.75e+2)-phi_dot.*t3.*t16.*t31.*t65.*(4.0./3.75e+2);
et200 = psi_dot.*t16.*t18.*t24.*t92.*(-2.25e-3)-t3.*t24.*t31.*t92.*zeta_dot.*8.25e-3-phi_dot.*t16.*t18.*t24.*t31.*t92.*(3.0./5.0e+2)-t3.*t16.*t18.*t24.*t92.*zeta_dot.*1.05e-2;
et201 = -t119+t226+t270-t290+t303+t349+t375+t530-t644+t747-t800+t871-t921+t968+t1045-t1097-t1134-t1150+t1164+t1242+t1328+t1401+t1406+t1507+t1536+t1585+t1620+t1671+t1747-t1775+t1845-t1921-t1990+t2046+t2054-t2104-t2162-psi_dot.*t26.*t31.*6.75e-3-t11.*t16.*zeta_dot.*(2.1e+1./1.0e+3)-psi_dot.*t3.*t16.*t26.*(3.0./1.0e+3)-psi_dot.*t16.*t18.*t26.*1.05e-2+t11.*t18.*t31.*zeta_dot.*2.55e-2+t11.*t16.*t92.*zeta_dot.*4.5e-3-phi_dot.*t3.*t16.*t31.*t67.*(4.0./3.75e+2)-phi_dot.*t26.*t47.*t73.*t92.*1.05e-2+psi_dot.*t16.*t18.*t26.*t92.*2.25e-3;
et202 = t3.*t26.*t31.*t92.*zeta_dot.*(-1.275e-2)-(t3.*t11.*t26.*t31.*t92.*zeta_dot)./3.75e+2-phi_dot.*t11.*t16.*t18.*t26.*t31.*t92.*(2.0./3.75e+2);
et203 = -t120+t228+t271-t291+t303+t349+t377+t531-t645+t749-t801+t873+t922+t970+t1046-t1098-t1135-t1151+t1165+t1243+t1508+t1537+t1569+t1586-t1748+t1772+t1776+t1807-t1846+t1922+t1991+t2023-t2055+t2105+t2137+t2163-psi_dot.*t27.*t31.*6.75e-3-t12.*t16.*zeta_dot.*(2.1e+1./1.0e+3)-phi_dot.*t27.*t73.*t92.*1.05e-2-psi_dot.*t3.*t16.*t27.*(3.0./1.0e+3)-psi_dot.*t16.*t18.*t27.*1.05e-2-psi_dot.*t27.*t31.*t92.*1.05e-2+t12.*t18.*t31.*zeta_dot.*2.55e-2-t12.*t16.*t92.*zeta_dot.*4.5e-3-t16.*t68.*t92.*zeta_dot.*(2.0./3.75e+2)-phi_dot.*t3.*t16.*t31.*t68.*(4.0./3.75e+2);
et204 = psi_dot.*t16.*t18.*t27.*t92.*(-2.25e-3)+t3.*t27.*t31.*t92.*zeta_dot.*1.275e-2-t3.*t16.*t18.*t27.*t92.*zeta_dot.*1.05e-2;
et205 = -t122+t232+t272-t292+t303+t349+t378+t532-t647+t750-t803+t874+t923+t972+t1048-t1100-t1136-t1152-t1245+t1401+t1408+t1510+t1538-t1588+t1620+t1749-t1777+t1847-t1923-t1992+t2056-t2106+t2138-t2164-psi_dot.*t29.*t31.*6.75e-3+t14.*t16.*zeta_dot.*(2.1e+1./1.0e+3)-phi_dot.*t29.*t73.*t92.*1.05e-2-psi_dot.*t3.*t16.*t29.*(3.0./1.0e+3)+psi_dot.*t16.*t18.*t29.*1.05e-2-psi_dot.*t29.*t31.*t92.*1.05e-2+t14.*t18.*t31.*zeta_dot.*2.55e-2+t14.*t16.*t92.*zeta_dot.*4.5e-3-phi_dot.*t16.*t18.*t29.*t31.*1.05e-2-phi_dot.*t3.*t16.*t31.*t70.*(4.0./3.75e+2);
et206 = psi_dot.*t16.*t18.*t29.*t92.*2.25e-3-t3.*t29.*t31.*t92.*zeta_dot.*1.275e-2-t3.*t16.*t18.*t29.*t92.*zeta_dot.*1.05e-2-(t3.*t14.*t29.*t31.*t92.*zeta_dot)./3.75e+2-phi_dot.*t14.*t16.*t18.*t29.*t31.*t92.*(2.0./3.75e+2);
et207 = -t123+t234+t273-t293+t303+t349+t380+t533-t648+t752-t804+t876-t924+t974+t1049-t1101-t1137-t1153-t1246+t1331+t1511+t1539+t1569-t1589+t1674-t1750+t1774+t1778+t1807-t1848+t1924+t1993+t2025+t2049-t2057+t2107+t2165-psi_dot.*t30.*t31.*6.75e-3+t15.*t16.*zeta_dot.*(2.1e+1./1.0e+3)-psi_dot.*t3.*t16.*t30.*(3.0./1.0e+3)+psi_dot.*t16.*t18.*t30.*1.05e-2+t15.*t18.*t31.*zeta_dot.*2.55e-2-t15.*t16.*t92.*zeta_dot.*4.5e-3-t16.*t71.*t92.*zeta_dot.*(2.0./3.75e+2)-phi_dot.*t16.*t18.*t30.*t31.*1.05e-2-phi_dot.*t3.*t16.*t31.*t71.*(4.0./3.75e+2)-phi_dot.*t30.*t47.*t73.*t92.*1.05e-2;
et208 = psi_dot.*t16.*t18.*t30.*t92.*(-2.25e-3)+t3.*t30.*t31.*t92.*zeta_dot.*1.275e-2;
mt1 = [0.0,0.0,0.0,0.0,0.0,0.0,0.0,0.0,0.0,0.0,0.0,0.0,0.0,0.0,0.0,0.0,0.0,0.0,0.0,0.0,0.0,0.0,0.0,0.0,0.0,0.0,0.0,0.0,0.0,0.0,0.0,0.0,0.0,0.0,0.0,0.0,0.0,0.0,0.0,0.0,0.0,0.0,0.0,0.0,0.0,0.0,0.0,0.0,0.0,0.0,0.0,0.0,0.0,0.0,0.0,0.0,0.0,0.0,0.0,0.0,0.0,0.0,0.0,0.0,0.0,0.0,0.0,0.0,0.0,0.0,0.0,0.0,0.0,0.0,0.0,0.0,0.0,0.0,0.0,0.0,0.0,0.0,0.0,0.0,0.0,0.0,0.0,0.0,0.0,0.0,et1+et2+et3+et4+et5+et6+et7+et8+et9,et24+et25+et26+et27+et28+et29+et30+et31+et32,0.0,et56+et57+et58+et59+et60+et61+et62+et63+et64+et65+et66+et67+et68+et69+et70+et71+et72+et73+et74+et75+et76+et77+et78+et79+et80+et81+et82+et83+et84+et85+et86+et87+et88+et89+et90+et91+et92+et93+et94+et95+et96+et97+et98,et140+et141+et142+et143+et144+et145+et146+et147+et148+et149+et150,et171+et172+et173+et174+et175+et176+et177+et178+et179+et180+et181+et182+et183];
mt2 = [-t112-t165+t187+t212+t370+t522+t584+t633-t637+t793+t1038-t1090+t1154-t1235+t1410+t1500-t1578+t3.*t213+t4.*t16.*zeta_dot.*(2.1e+1./1.0e+3)-psi_dot.*t16.*t18.*t19.*(2.1e+1./1.0e+3)-psi_dot.*t3.*t16.*t60.*(4.0./3.75e+2)-t4.*t18.*t31.*zeta_dot.*(3.0./1.0e+2)-t18.*t31.*t60.*zeta_dot.*(4.0./3.75e+2)-phi_dot.*t3.*t16.*t19.*t31.*(3.0./5.0e+2),et193+et194,et195+et196,0.0,0.0,0.0];
mt3 = [-t115-t166+t187+t218+t373+t523+t584+t634-t640+t796+t1041-t1093+t1238+t1411+t1503+t1581+t3.*t219-t7.*t16.*zeta_dot.*(2.1e+1./1.0e+3)+psi_dot.*t16.*t18.*t22.*(2.1e+1./1.0e+3)-psi_dot.*t3.*t16.*t63.*(4.0./3.75e+2)-t7.*t18.*t31.*zeta_dot.*(3.0./1.0e+2)-t18.*t31.*t63.*zeta_dot.*(4.0./3.75e+2)-phi_dot.*t3.*t16.*t22.*t31.*(3.0./5.0e+2)-phi_dot.*t16.*t18.*t22.*t31.*(2.1e+1./1.0e+3),et197+et198,et199+et200,0.0,0.0,0.0];
mt4 = [-t118-t167+t187+t224+t376-t528+t584-t635-t643+t799+t1044-t1096+t1241+t1412+t1506+t1584+t3.*t225-t10.*t16.*zeta_dot.*(2.1e+1./1.0e+3)+psi_dot.*t16.*t18.*t25.*(2.1e+1./1.0e+3)-psi_dot.*t3.*t16.*t66.*(4.0./3.75e+2)+t10.*t18.*t31.*zeta_dot.*(3.0./2.5e+2)-t18.*t31.*t66.*zeta_dot.*(4.0./3.75e+2)-phi_dot.*t3.*t16.*t25.*t31.*(3.0./5.0e+2)-phi_dot.*t16.*t18.*t25.*t31.*(2.1e+1./1.0e+3),et201+et202,et203+et204,0.0,0.0,0.0];
mt5 = [-t121-t168+t187+t230+t379-t529+t584-t636-t646+t802+t1047-t1099+t1157-t1244+t1413+t1509-t1587+t3.*t231+t13.*t16.*zeta_dot.*(2.1e+1./1.0e+3)-psi_dot.*t16.*t18.*t28.*(2.1e+1./1.0e+3)-psi_dot.*t3.*t16.*t69.*(4.0./3.75e+2)+t13.*t18.*t31.*zeta_dot.*(3.0./2.5e+2)-t18.*t31.*t69.*zeta_dot.*(4.0./3.75e+2)-phi_dot.*t3.*t16.*t28.*t31.*(3.0./5.0e+2),et205+et206,et207+et208,0.0,0.0,0.0,et10+et11+et12+et13+et14+et15+et16,et33+et34+et35+et36+et37+et38+et39,et47+et48+et49+et50+et51,et99+et100+et101+et102+et103+et104+et105+et106+et107+et108+et109+et110+et111+et112,et151+et152+et153+et154+et155+et156+et157+et158+et159+et160+et161,et184+et185+et186+et187+et188+et189+et190];
mt6 = [t151+t159+t173-t352+t394-t478+t491+t671-t805-t842-t1066-psi_dot.*t3.*t19.*(2.1e+1./1.0e+3)-psi_dot.*t18.*t19.*(3.0./5.0e+2)-phi_dot.*t4.*t16.*t47.*(2.1e+1./1.0e+3)-phi_dot.*t3.*t4.*t16.*t18.*(3.0./5.0e+2)];
mt7 = [t136-t161+t174+t395-t479+t672-t700-t806+t841-t909+t935-t1067+t1174+t1392+t1393+t1428+t1460+t1629+t1783+t1797+t1816-t1962+psi_dot.*t3.*t20.*1.05e-2+psi_dot.*t18.*t20.*(3.0./1.0e+3)-psi_dot.*t18.*t61.*(2.0./3.75e+2)-phi_dot.*t5.*t16.*t47.*(2.1e+1./1.0e+3)+psi_dot.*t3.*t20.*t92.*2.25e-3-t20.*t47.*t92.*zeta_dot.*1.05e-2-phi_dot.*t3.*t5.*t16.*t18.*(3.0./5.0e+2)-phi_dot.*t3.*t16.*t18.*t20.*6.75e-3-phi_dot.*t5.*t16.*t47.*t92.*4.5e-3-t3.*t18.*t20.*t92.*zeta_dot.*(3.0./1.0e+3)-phi_dot.*t3.*t16.*t18.*t20.*t92.*1.05e-2-(phi_dot.*t3.*t5.*t20.*t31.*t92)./3.75e+2];
mt8 = [t136-t162+t175+t396-t480+t673-t702-t807+t843-t910-t936+t989-t1068-t1394-t1429-t1461+t1540+t1600-t1630+t1692+t1729-t1784-t1798-t1817+t1886+t1963+t2027+psi_dot.*t3.*t21.*1.05e-2+psi_dot.*t18.*t21.*(3.0./1.0e+3)-psi_dot.*t18.*t62.*(2.0./3.75e+2)-phi_dot.*t6.*t16.*t47.*(2.1e+1./1.0e+3)-psi_dot.*t3.*t21.*t92.*2.25e-3-phi_dot.*t3.*t6.*t16.*t18.*(3.0./5.0e+2)-phi_dot.*t3.*t16.*t18.*t21.*6.75e-3,0.0,0.0,0.0];
mt9 = [t152+t159+t176-t354-t397-t481+t494-t674-t808-t845-t1069+t1206+psi_dot.*t3.*t22.*(2.1e+1./1.0e+3)-psi_dot.*t18.*t22.*(3.0./5.0e+2)-phi_dot.*t3.*t7.*t16.*t18.*(3.0./5.0e+2)];
mt10 = [t136-t163+t177-t398-t482-t675-t708-t809+t844-t911-t937-t1070+t1174+t1207+t1392+t1395+t1430+t1462+t1631+t1693+t1785+t1801+t1818-t1964+t2028-psi_dot.*t3.*t23.*1.05e-2+psi_dot.*t18.*t23.*(3.0./1.0e+3)-psi_dot.*t18.*t64.*(2.0./3.75e+2)+psi_dot.*t3.*t23.*t92.*2.25e-3-phi_dot.*t3.*t8.*t16.*t18.*(3.0./5.0e+2)-phi_dot.*t3.*t16.*t18.*t23.*6.75e-3-phi_dot.*t8.*t16.*t47.*t92.*4.5e-3-t3.*t18.*t23.*t92.*zeta_dot.*(3.0./1.0e+3)-(phi_dot.*t3.*t8.*t23.*t31.*t92)./3.75e+2];
mt11 = [t136-t164+t178-t399-t483-t676-t710-t810+t846-t912+t938+t989-t1071+t1208-t1396-t1431-t1463+t1540+t1602-t1632+t1733-t1786-t1802-t1819+t1888+t1965-psi_dot.*t3.*t24.*1.05e-2+psi_dot.*t18.*t24.*(3.0./1.0e+3)-psi_dot.*t18.*t65.*(2.0./3.75e+2)-psi_dot.*t3.*t24.*t92.*2.25e-3-t24.*t47.*t92.*zeta_dot.*1.05e-2-phi_dot.*t3.*t9.*t16.*t18.*(3.0./5.0e+2)-phi_dot.*t3.*t16.*t18.*t24.*6.75e-3-phi_dot.*t3.*t16.*t18.*t24.*t92.*1.05e-2,0.0,0.0,0.0];
mt12 = [-t153+t159+t179+t356-t400-t484+t497-t677-t811-t848-t1072+t1209+psi_dot.*t3.*t25.*(2.1e+1./1.0e+3)-psi_dot.*t18.*t25.*(3.0./5.0e+2)-phi_dot.*t3.*t10.*t16.*t18.*(3.0./5.0e+2)];
mt13 = [t136+t180+t282-t401-t485-t678+t716-t812+t847-t913-t939-t1073+t1174+t1210+t1392+t1397+t1432+t1466+t1633+t1695+t1787-t1803+t1820-t1966+t2030-psi_dot.*t3.*t26.*1.05e-2+psi_dot.*t18.*t26.*(3.0./1.0e+3)-psi_dot.*t18.*t67.*(2.0./3.75e+2)+psi_dot.*t3.*t26.*t92.*2.25e-3-phi_dot.*t3.*t11.*t16.*t18.*(3.0./5.0e+2)-phi_dot.*t3.*t16.*t18.*t26.*6.75e-3-phi_dot.*t11.*t16.*t47.*t92.*4.5e-3-t3.*t18.*t26.*t92.*zeta_dot.*(3.0./1.0e+3)-(phi_dot.*t3.*t11.*t26.*t31.*t92)./3.75e+2];
mt14 = [t136+t181+t283-t402-t486-t679+t718-t813+t849-t914+t940+t989-t1074+t1211-t1398-t1433-t1467+t1540+t1604-t1634+t1737-t1788+t1804-t1821+t1890+t1967-psi_dot.*t3.*t27.*1.05e-2+psi_dot.*t18.*t27.*(3.0./1.0e+3)-psi_dot.*t18.*t68.*(2.0./3.75e+2)-psi_dot.*t3.*t27.*t92.*2.25e-3-t27.*t47.*t92.*zeta_dot.*1.05e-2-phi_dot.*t3.*t12.*t16.*t18.*(3.0./5.0e+2)-phi_dot.*t3.*t16.*t18.*t27.*6.75e-3-phi_dot.*t3.*t16.*t18.*t27.*t92.*1.05e-2,0.0,0.0,0.0];
mt15 = [-t154+t159+t182+t358+t403-t487+t500+t680-t814-t851-t1075-psi_dot.*t3.*t28.*(2.1e+1./1.0e+3)-psi_dot.*t18.*t28.*(3.0./5.0e+2)-phi_dot.*t13.*t16.*t47.*(2.1e+1./1.0e+3)-phi_dot.*t3.*t13.*t16.*t18.*(3.0./5.0e+2)];
mt16 = [t136+t183+t284+t404-t488+t681+t720-t815+t850-t915+t941-t1076+t1174+t1392+t1399+t1434+t1470+t1635+t1789-t1805+t1822-t1968+psi_dot.*t3.*t29.*1.05e-2+psi_dot.*t18.*t29.*(3.0./1.0e+3)-psi_dot.*t18.*t70.*(2.0./3.75e+2)-phi_dot.*t14.*t16.*t47.*(2.1e+1./1.0e+3)+psi_dot.*t3.*t29.*t92.*2.25e-3-t29.*t47.*t92.*zeta_dot.*1.05e-2-phi_dot.*t3.*t14.*t16.*t18.*(3.0./5.0e+2)-phi_dot.*t3.*t16.*t18.*t29.*6.75e-3-phi_dot.*t14.*t16.*t47.*t92.*4.5e-3-t3.*t18.*t29.*t92.*zeta_dot.*(3.0./1.0e+3)-phi_dot.*t3.*t16.*t18.*t29.*t92.*1.05e-2-(phi_dot.*t3.*t14.*t29.*t31.*t92)./3.75e+2];
mt17 = [t136+t184+t285+t405-t489+t682+t722-t816+t852-t916-t942+t989-t1077-t1400-t1435-t1471+t1540+t1606-t1636+t1698+t1741-t1790+t1806-t1823+t1892+t1969+t2033+psi_dot.*t3.*t30.*1.05e-2+psi_dot.*t18.*t30.*(3.0./1.0e+3)-psi_dot.*t18.*t71.*(2.0./3.75e+2)-phi_dot.*t15.*t16.*t47.*(2.1e+1./1.0e+3)-psi_dot.*t3.*t30.*t92.*2.25e-3-phi_dot.*t3.*t15.*t16.*t18.*(3.0./5.0e+2)-phi_dot.*t3.*t16.*t18.*t30.*6.75e-3,0.0,0.0,0.0,et17+et18+et19+et20+et21+et22+et23,et40+et41+et42+et43+et44+et45+et46,et52+et53+et54+et55,et113+et114+et115+et116+et117+et118+et119+et120+et121+et122+et123,et162+et163+et164+et165+et166+et167+et168+et169+et170,et191+et192];
mt18 = [-t124+t160-t169+t185+t188-t248+t325+t342-t434+t534-t684-phi_dot.*t3.*t16.*t48.*(2.0./3.75e+2),-t125+t150+t190+t274-t294+t302+t316+t361+t438-t568+t692+t733+t925+t1436+t1492+t1728+t1791-phi_dot.*t20.*t31.*6.75e-3-t18.*t61.*zeta_dot.*(2.0./3.75e+2)-phi_dot.*t20.*t31.*t92.*1.05e-2,-t126+t150+t192+t275-t295+t302+t317+t362+t439-t570+t694+t734-t926+t1317-t1437-t1493-t1730-t1792-phi_dot.*t21.*t31.*6.75e-3-t18.*t62.*zeta_dot.*(2.0./3.75e+2),0.0,0.0,0.0,-t127+t160-t170+t185+t194-t249+t326+t344+t435+t535+t686-phi_dot.*t3.*t16.*t51.*(2.0./3.75e+2)];
mt19 = [-t128+t150+t196+t276-t296+t302+t318+t363-t440-t572-t696+t735-t927+t1318+t1438+t1494+t1732+t1793-phi_dot.*t23.*t31.*6.75e-3-t18.*t64.*zeta_dot.*(2.0./3.75e+2),-t129+t150+t198+t277-t297+t302+t319+t364-t441-t574-t698+t736+t928-t1439-t1495-t1734-t1794-phi_dot.*t24.*t31.*6.75e-3-t18.*t65.*zeta_dot.*(2.0./3.75e+2)-phi_dot.*t24.*t31.*t92.*1.05e-2,0.0,0.0,0.0,-t130+t160-t171+t185+t200-t250+t327+t346+t436+t536+t688-phi_dot.*t3.*t16.*t54.*(2.0./3.75e+2)];
mt20 = [-t131+t150+t202+t278-t298+t302+t320+t365-t442-t576-t704+t737-t929+t1320+t1440+t1496+t1736+t1795-phi_dot.*t26.*t31.*6.75e-3-t18.*t67.*zeta_dot.*(2.0./3.75e+2),-t132+t150+t204+t279-t299+t302+t321+t366-t443-t578-t706+t738+t930-t1441-t1497-t1738-t1796-phi_dot.*t27.*t31.*6.75e-3-t18.*t68.*zeta_dot.*(2.0./3.75e+2)-phi_dot.*t27.*t31.*t92.*1.05e-2,0.0,0.0,0.0,-t133+t160-t172+t185+t206-t251+t328+t348-t437+t537-t690-phi_dot.*t3.*t16.*t57.*(2.0./3.75e+2)];
mt21 = [-t134+t150+t208+t280-t300+t302+t322+t367+t444-t580+t712+t739+t931+t1442+t1498+t1740+t1799-phi_dot.*t29.*t31.*6.75e-3-t18.*t70.*zeta_dot.*(2.0./3.75e+2)-phi_dot.*t29.*t31.*t92.*1.05e-2,-t135+t150+t210+t281-t301+t302+t323+t368+t445-t582+t714+t740-t932+t1323-t1443-t1499-t1742-t1800-phi_dot.*t30.*t31.*6.75e-3-t18.*t71.*zeta_dot.*(2.0./3.75e+2),0.0,0.0,0.0];
mt22 = [-phi_dot.*(t4.*t723.*(3.0./5.0e+1)-t16.*t17.*t19.*(3.0./5.0e+1))+th11_dot.*(t19.*t360.*(3.0./5.0e+1)-t2.*t4.*t16.*(3.0./5.0e+1))+zeta_dot.*((t2.*t990)./1.0e+2+t2.*t19.*t31.*(3.0./1.0e+2)-t4.*t16.*t88.*(3.0./1.0e+2))-psi_dot.*t4.*t724.*(3.0./5.0e+1),-phi_dot.*(t4.*t360.*(3.0./5.0e+1)+t2.*t16.*t19.*(3.0./5.0e+1))-th11_dot.*(t19.*t723.*(3.0./5.0e+1)+t4.*t16.*t17.*(3.0./5.0e+1))+zeta_dot.*((t17.*t990)./1.0e+2+t17.*t19.*t31.*(3.0./1.0e+2)-t4.*t16.*t90.*(3.0./1.0e+2))+psi_dot.*t4.*t359.*(3.0./5.0e+1)];
mt23 = [th11_dot.*(t4.*t31.*(3.0./5.0e+1)+t3.*t16.*t19.*(3.0./5.0e+1))+zeta_dot.*(t16.*t19.*(3.0./5.0e+1)+t3.*t4.*t31.*(3.0./5.0e+1))+psi_dot.*t4.*t16.*t18.*(3.0./5.0e+1)];
mt24 = [t112+t165+t324+t350-t370-t522-t633+t637+t658+t742-t793+t866+t1090+t1235-t1410+t1578-psi_dot.*t4.*t31.*(3.0./5.0e+2)-t19.*t31.*th11_dot.*(2.1e+1./1.0e+3)-phi_dot.*t4.*t47.*t73.*(3.0./5.0e+2)+psi_dot.*t3.*t4.*t16.*(3.0./1.0e+2)+t3.*t4.*t16.*th11_dot.*(2.1e+1./1.0e+3)+t4.*t16.*t18.*th11_dot.*(3.0./5.0e+2)-t16.*t18.*t19.*th11_dot.*(3.0./1.0e+2)-t3.*t19.*t31.*zeta_dot.*(2.1e+1./1.0e+3)-t18.*t19.*t31.*zeta_dot.*(3.0./5.0e+2)-phi_dot.*t16.*t18.*t19.*t31.*(2.1e+1./1.0e+3)-phi_dot.*t4.*t19.*t47.*t73.*(4.0./3.75e+2)];
mt25 = [-t151-t173+t352-t394+t478+t621-t671+t805+t842+t1066+t1203-psi_dot.*t4.*t18.*(3.0./1.0e+2)-psi_dot.*t18.*t60.*(4.0./3.75e+2)+t3.*t4.*th11_dot.*(3.0./5.0e+2)-t3.*t19.*th11_dot.*(3.0./1.0e+2)-t4.*t18.*th11_dot.*(2.1e+1./1.0e+3),t124+t150+t169+t248+t302+t434+t684+t725+t19.*th11_dot.*(2.1e+1./1.0e+3)-phi_dot.*t4.*t31.*(3.0./5.0e+2)-phi_dot.*t31.*t75.*(2.0./3.75e+2)-t18.*t48.*zeta_dot.*(2.0./3.75e+2)-phi_dot.*t3.*t16.*t19.*(3.0./5.0e+2),0.0,0.0,0.0,0.0,0.0,0.0,0.0,0.0,0.0,0.0,0.0,0.0,0.0,0.0,0.0,0.0,0.0,0.0,0.0,0.0,0.0,0.0,0.0,0.0];
mt26 = [-psi_dot.*(t5.*t724.*(3.0./5.0e+1)+t20.*t92.*t360.*(3.0./1.0e+2))-zeta_dot.*(t20.*t2148.*(3.0./5.0e+1)+t5.*t16.*t88.*(3.0./5.0e+1))-phi_dot.*(t5.*t723.*(3.0./5.0e+1)+t20.*t2178.*(3.0./5.0e+1))+th12_dot.*(t20.*t360.*(3.0./5.0e+1)+t5.*t2179.*(3.0./5.0e+1)),psi_dot.*(t5.*t359.*(3.0./5.0e+1)+t20.*t92.*t723.*(3.0./1.0e+2))-zeta_dot.*(t20.*t2149.*(3.0./5.0e+1)+t5.*t16.*t90.*(3.0./5.0e+1))-phi_dot.*(t5.*t360.*(3.0./5.0e+1)-t20.*t2179.*(3.0./5.0e+1))-th12_dot.*(t20.*t723.*(3.0./5.0e+1)-t5.*t2178.*(3.0./5.0e+1))];
mt27 = [-th12_dot.*(t5.*t1645.*(3.0./5.0e+1)-t3.*t16.*t20.*(3.0./5.0e+1))-t16.*t20.*zeta_dot.*(3.0./1.0e+2)+psi_dot.*t5.*t16.*t18.*(3.0./5.0e+1)+t3.*t5.*t31.*zeta_dot.*(3.0./5.0e+1)-psi_dot.*t3.*t16.*t20.*t92.*(3.0./1.0e+2)+t18.*t20.*t31.*t92.*zeta_dot.*(3.0./1.0e+2),et124+et125];
mt28 = [t161-t174-t395+t479+t490+t622-t672+t700+t806-t841+t909-t935+t989+t1067+t1138+t1204-t1393-t1428-t1460+t1540+t1599-t1629+t1691+t1727-t1783-t1797-t1816+t1885+t1962+t2026-psi_dot.*t5.*t18.*1.65e-2-t3.*t5.*th12_dot.*(3.0./1.0e+3)-t3.*t20.*th12_dot.*1.65e-2+t5.*t18.*th12_dot.*1.05e-2+psi_dot.*t3.*t20.*t92.*8.25e-3+t5.*t18.*t92.*th12_dot.*1.05e-2];
mt29 = [t125+t160+t185-t274+t294-t316-t361-t438+t446+t538+t568-t692-t925+t1316-t1436-t1492-t1728-t1791+t20.*th12_dot.*(2.1e+1./1.0e+3)-phi_dot.*t5.*t31.*(3.0./5.0e+2)-t5.*t92.*th12_dot.*(3.0./1.0e+3)+t20.*t92.*th12_dot.*4.5e-3-phi_dot.*t3.*t16.*t61.*(2.0./3.75e+2),0.0,0.0,0.0,0.0,0.0,0.0,0.0,0.0,0.0,0.0,0.0,0.0,0.0,0.0,0.0,0.0,0.0,0.0,0.0,0.0,0.0,0.0,0.0,0.0];
mt30 = [-psi_dot.*(t6.*t724.*(3.0./5.0e+1)-t21.*t92.*t360.*(3.0./1.0e+2))-zeta_dot.*(t21.*t2175.*(3.0./5.0e+1)+t6.*t16.*t88.*(3.0./5.0e+1))-phi_dot.*(t6.*t723.*(3.0./5.0e+1)+t21.*t2177.*(3.0./5.0e+1))+th13_dot.*(t21.*t360.*(3.0./5.0e+1)+t6.*t2180.*(3.0./5.0e+1)),psi_dot.*(t6.*t359.*(3.0./5.0e+1)-t21.*t92.*t723.*(3.0./1.0e+2))-zeta_dot.*(t21.*t2176.*(3.0./5.0e+1)+t6.*t16.*t90.*(3.0./5.0e+1))-phi_dot.*(t6.*t360.*(3.0./5.0e+1)-t21.*t2180.*(3.0./5.0e+1))-th13_dot.*(t21.*t723.*(3.0./5.0e+1)-t6.*t2177.*(3.0./5.0e+1))];
mt31 = [-th13_dot.*(t6.*t1840.*(3.0./5.0e+1)-t3.*t16.*t21.*(3.0./5.0e+1))-t16.*t21.*zeta_dot.*(3.0./1.0e+2)+psi_dot.*t6.*t16.*t18.*(3.0./5.0e+1)+t3.*t6.*t31.*zeta_dot.*(3.0./5.0e+1)+psi_dot.*t3.*t16.*t21.*t92.*(3.0./1.0e+2)-t18.*t21.*t31.*t92.*zeta_dot.*(3.0./1.0e+2),et126+et127];
mt32 = [t162-t175-t396+t480+t492+t623-t673+t702+t807-t843+t910+t936+t1068+t1139+t1174+t1205+t1392+t1394+t1429+t1461+t1630+t1784+t1798+t1817-t1963-psi_dot.*t6.*t18.*1.65e-2-t3.*t6.*th13_dot.*(3.0./1.0e+3)-t3.*t21.*th13_dot.*1.65e-2+t6.*t18.*th13_dot.*1.05e-2-psi_dot.*t3.*t21.*t92.*8.25e-3-t6.*t18.*t92.*th13_dot.*1.05e-2-t21.*t47.*t92.*zeta_dot.*1.05e-2-phi_dot.*t6.*t16.*t47.*t92.*4.5e-3-t3.*t18.*t21.*t92.*zeta_dot.*(3.0./1.0e+3)-phi_dot.*t3.*t16.*t18.*t21.*t92.*1.05e-2-(phi_dot.*t3.*t6.*t21.*t31.*t92)./3.75e+2];
mt33 = [t126+t160+t185-t275+t295-t317-t362-t439+t447+t539+t570-t694+t926+t1437+t1493+t1730+t1792+t21.*th13_dot.*(2.1e+1./1.0e+3)-phi_dot.*t6.*t31.*(3.0./5.0e+2)+t6.*t92.*th13_dot.*(3.0./1.0e+3)-t21.*t92.*th13_dot.*4.5e-3-phi_dot.*t3.*t16.*t62.*(2.0./3.75e+2)-phi_dot.*t21.*t31.*t92.*1.05e-2,0.0,0.0,0.0,0.0,0.0,0.0,0.0,0.0,0.0,0.0,0.0,0.0,0.0,0.0,0.0,0.0,0.0,0.0,0.0,0.0,0.0,0.0,0.0,0.0,0.0,0.0,0.0,0.0,0.0,0.0,0.0,0.0,0.0,0.0,0.0,0.0,0.0,0.0,0.0,0.0,0.0,0.0,0.0,0.0,0.0,0.0,0.0,0.0,0.0,0.0,0.0,0.0,0.0,0.0,0.0,0.0,0.0,0.0,0.0,0.0,0.0,0.0,0.0,0.0,0.0,0.0,0.0,0.0,0.0,0.0,0.0,0.0,0.0,0.0,0.0,0.0,0.0,0.0,0.0,0.0,0.0,0.0,0.0,0.0,0.0,0.0,0.0,0.0,0.0,0.0,0.0,0.0,0.0,0.0,0.0,0.0,0.0,0.0,0.0,0.0,0.0];
mt34 = [0.0,0.0,0.0,0.0,0.0,0.0,0.0,0.0,0.0,0.0,0.0,0.0,0.0,-phi_dot.*(t7.*t723.*(3.0./5.0e+1)-t16.*t17.*t22.*(3.0./5.0e+1))+th21_dot.*(t22.*t360.*(3.0./5.0e+1)-t2.*t7.*t16.*(3.0./5.0e+1))+zeta_dot.*((t2.*t991)./1.0e+2+t2.*t22.*t31.*(3.0./1.0e+2)-t7.*t16.*t88.*(3.0./1.0e+2))-psi_dot.*t7.*t724.*(3.0./5.0e+1),-phi_dot.*(t7.*t360.*(3.0./5.0e+1)+t2.*t16.*t22.*(3.0./5.0e+1))-th21_dot.*(t22.*t723.*(3.0./5.0e+1)+t7.*t16.*t17.*(3.0./5.0e+1))+zeta_dot.*((t17.*t991)./1.0e+2+t17.*t22.*t31.*(3.0./1.0e+2)-t7.*t16.*t90.*(3.0./1.0e+2))+psi_dot.*t7.*t359.*(3.0./5.0e+1)];
mt35 = [th21_dot.*(t7.*t31.*(3.0./5.0e+1)+t3.*t16.*t22.*(3.0./5.0e+1))+zeta_dot.*(t16.*t22.*(3.0./5.0e+1)+t3.*t7.*t31.*(3.0./5.0e+1))+psi_dot.*t7.*t16.*t18.*(3.0./5.0e+1),t115+t166+t324+t350-t373-t523-t634+t640+t660+t745-t796+t869+t1093+t1155-t1238-t1411-t1581+t31.*t435-psi_dot.*t7.*t31.*(3.0./5.0e+2)+t22.*t31.*th21_dot.*(2.1e+1./1.0e+3)-phi_dot.*t7.*t47.*t73.*(3.0./5.0e+2)+psi_dot.*t3.*t7.*t16.*(3.0./1.0e+2)-t3.*t7.*t16.*th21_dot.*(2.1e+1./1.0e+3)+t7.*t16.*t18.*th21_dot.*(3.0./5.0e+2)-t16.*t18.*t22.*th21_dot.*(3.0./1.0e+2)-t18.*t22.*t31.*zeta_dot.*(3.0./5.0e+2)-phi_dot.*t7.*t22.*t47.*t73.*(4.0./3.75e+2)];
mt36 = [-t152-t176+t354+t397+t481+t624+t674+t808+t845+t1069-psi_dot.*t7.*t18.*(3.0./1.0e+2)-psi_dot.*t18.*t63.*(4.0./3.75e+2)+t3.*t7.*th21_dot.*(3.0./5.0e+2)-t3.*t22.*th21_dot.*(3.0./1.0e+2)+t7.*t18.*th21_dot.*(2.1e+1./1.0e+3)-phi_dot.*t7.*t16.*t47.*(2.1e+1./1.0e+3),t127+t150+t170+t249+t302-t435-t686+t726-t22.*th21_dot.*(2.1e+1./1.0e+3)-phi_dot.*t7.*t31.*(3.0./5.0e+2)-phi_dot.*t31.*t78.*(2.0./3.75e+2)-t18.*t51.*zeta_dot.*(2.0./3.75e+2)-phi_dot.*t3.*t16.*t22.*(3.0./5.0e+2),0.0,0.0,0.0,0.0,0.0,0.0,0.0,0.0,0.0,0.0,0.0,0.0,0.0,0.0,0.0,0.0,0.0,0.0,0.0,0.0,0.0,0.0,0.0,0.0];
mt37 = [-psi_dot.*(t8.*t724.*(3.0./5.0e+1)+t23.*t92.*t360.*(3.0./1.0e+2))-zeta_dot.*(t23.*t2148.*(3.0./5.0e+1)+t8.*t16.*t88.*(3.0./5.0e+1))-phi_dot.*(t8.*t723.*(3.0./5.0e+1)+t23.*t2178.*(3.0./5.0e+1))+th22_dot.*(t23.*t360.*(3.0./5.0e+1)+t8.*t2179.*(3.0./5.0e+1)),psi_dot.*(t8.*t359.*(3.0./5.0e+1)+t23.*t92.*t723.*(3.0./1.0e+2))-zeta_dot.*(t23.*t2149.*(3.0./5.0e+1)+t8.*t16.*t90.*(3.0./5.0e+1))-phi_dot.*(t8.*t360.*(3.0./5.0e+1)-t23.*t2179.*(3.0./5.0e+1))-th22_dot.*(t23.*t723.*(3.0./5.0e+1)-t8.*t2178.*(3.0./5.0e+1))];
mt38 = [-th22_dot.*(t8.*t1645.*(3.0./5.0e+1)-t3.*t16.*t23.*(3.0./5.0e+1))-t16.*t23.*zeta_dot.*(3.0./1.0e+2)+psi_dot.*t8.*t16.*t18.*(3.0./5.0e+1)+t3.*t8.*t31.*zeta_dot.*(3.0./5.0e+1)-psi_dot.*t3.*t16.*t23.*t92.*(3.0./1.0e+2)+t18.*t23.*t31.*t92.*zeta_dot.*(3.0./1.0e+2),et128+et129];
mt39 = [t163-t177+t398+t482+t493+t625+t675+t708+t809-t844+t911+t937+t989+t1070+t1140-t1395-t1430-t1462+t1540+t1601-t1631+t1731-t1785-t1801-t1818+t1887+t1964-psi_dot.*t8.*t18.*1.65e-2-t3.*t8.*th22_dot.*(3.0./1.0e+3)-t3.*t23.*th22_dot.*1.65e-2-t8.*t18.*th22_dot.*1.05e-2-phi_dot.*t8.*t16.*t47.*(2.1e+1./1.0e+3)+psi_dot.*t3.*t23.*t92.*8.25e-3+t8.*t18.*t92.*th22_dot.*1.05e-2-t23.*t47.*t92.*zeta_dot.*1.05e-2-phi_dot.*t3.*t16.*t18.*t23.*t92.*1.05e-2];
mt40 = [t128+t160+t185-t276+t296-t318-t363+t440+t448+t540+t572+t696+t927-t1438-t1494-t1732-t1793-t23.*th22_dot.*(2.1e+1./1.0e+3)-phi_dot.*t8.*t31.*(3.0./5.0e+2)-t8.*t92.*th22_dot.*(3.0./1.0e+3)+t23.*t92.*th22_dot.*4.5e-3-phi_dot.*t3.*t16.*t64.*(2.0./3.75e+2)-phi_dot.*t23.*t31.*t92.*1.05e-2,0.0,0.0,0.0,0.0,0.0,0.0,0.0,0.0,0.0,0.0,0.0,0.0,0.0,0.0,0.0,0.0,0.0,0.0,0.0,0.0,0.0,0.0,0.0,0.0];
mt41 = [-psi_dot.*(t9.*t724.*(3.0./5.0e+1)-t24.*t92.*t360.*(3.0./1.0e+2))-zeta_dot.*(t24.*t2175.*(3.0./5.0e+1)+t9.*t16.*t88.*(3.0./5.0e+1))-phi_dot.*(t9.*t723.*(3.0./5.0e+1)+t24.*t2177.*(3.0./5.0e+1))+th23_dot.*(t24.*t360.*(3.0./5.0e+1)+t9.*t2180.*(3.0./5.0e+1)),psi_dot.*(t9.*t359.*(3.0./5.0e+1)-t24.*t92.*t723.*(3.0./1.0e+2))-zeta_dot.*(t24.*t2176.*(3.0./5.0e+1)+t9.*t16.*t90.*(3.0./5.0e+1))-phi_dot.*(t9.*t360.*(3.0./5.0e+1)-t24.*t2180.*(3.0./5.0e+1))-th23_dot.*(t24.*t723.*(3.0./5.0e+1)-t9.*t2177.*(3.0./5.0e+1))];
mt42 = [-th23_dot.*(t9.*t1840.*(3.0./5.0e+1)-t3.*t16.*t24.*(3.0./5.0e+1))-t16.*t24.*zeta_dot.*(3.0./1.0e+2)+psi_dot.*t9.*t16.*t18.*(3.0./5.0e+1)+t3.*t9.*t31.*zeta_dot.*(3.0./5.0e+1)+psi_dot.*t3.*t16.*t24.*t92.*(3.0./1.0e+2)-t18.*t24.*t31.*t92.*zeta_dot.*(3.0./1.0e+2),et130+et131];
mt43 = [t164-t178+t399+t483+t495+t626+t676+t710+t810-t846+t912-t938+t1071+t1141+t1174+t1392+t1396+t1431+t1463+t1632+t1694+t1786+t1802+t1819-t1965+t2029-psi_dot.*t9.*t18.*1.65e-2-t3.*t9.*th23_dot.*(3.0./1.0e+3)-t3.*t24.*th23_dot.*1.65e-2-t9.*t18.*th23_dot.*1.05e-2-phi_dot.*t9.*t16.*t47.*(2.1e+1./1.0e+3)-psi_dot.*t3.*t24.*t92.*8.25e-3-t9.*t18.*t92.*th23_dot.*1.05e-2-phi_dot.*t9.*t16.*t47.*t92.*4.5e-3-t3.*t18.*t24.*t92.*zeta_dot.*(3.0./1.0e+3)-(phi_dot.*t3.*t9.*t24.*t31.*t92)./3.75e+2];
mt44 = [t129+t160+t185-t277+t297-t319-t364+t441+t449+t541+t574+t698-t928+t1319+t1439+t1495+t1734+t1794-t24.*th23_dot.*(2.1e+1./1.0e+3)-phi_dot.*t9.*t31.*(3.0./5.0e+2)+t9.*t92.*th23_dot.*(3.0./1.0e+3)-t24.*t92.*th23_dot.*4.5e-3-phi_dot.*t3.*t16.*t65.*(2.0./3.75e+2),0.0,0.0,0.0,0.0,0.0,0.0,0.0,0.0,0.0,0.0,0.0,0.0,0.0,0.0,0.0,0.0,0.0,0.0,0.0,0.0,0.0,0.0,0.0,0.0,0.0,0.0,0.0,0.0,0.0,0.0,0.0,0.0,0.0,0.0,0.0,0.0,0.0,0.0,0.0,0.0,0.0,0.0,0.0,0.0,0.0,0.0,0.0,0.0,0.0,0.0,0.0,0.0,0.0,0.0,0.0,0.0,0.0,0.0,0.0,0.0,0.0,0.0,0.0,0.0,0.0,0.0,0.0,0.0,0.0,0.0,0.0,0.0,0.0,0.0,0.0,0.0,0.0,0.0,0.0,0.0,0.0,0.0,0.0,0.0,0.0,0.0,0.0,0.0,0.0,0.0,0.0,0.0,0.0,0.0,0.0,0.0,0.0,0.0,0.0,0.0,0.0,0.0,0.0,0.0,0.0,0.0,0.0,0.0,0.0,0.0,0.0,0.0,0.0,0.0];
mt45 = [-phi_dot.*(t10.*t723.*(3.0./5.0e+1)-t16.*t17.*t25.*(3.0./5.0e+1))+th31_dot.*(t25.*t360.*(3.0./5.0e+1)-t2.*t10.*t16.*(3.0./5.0e+1))+zeta_dot.*((t2.*t992)./1.0e+2+t2.*t25.*t31.*(3.0./1.0e+2)-t10.*t16.*t88.*(3.0./1.0e+2))-psi_dot.*t10.*t724.*(3.0./5.0e+1),-phi_dot.*(t10.*t360.*(3.0./5.0e+1)+t2.*t16.*t25.*(3.0./5.0e+1))-th31_dot.*(t25.*t723.*(3.0./5.0e+1)+t10.*t16.*t17.*(3.0./5.0e+1))+zeta_dot.*((t17.*t992)./1.0e+2+t17.*t25.*t31.*(3.0./1.0e+2)-t10.*t16.*t90.*(3.0./1.0e+2))+psi_dot.*t10.*t359.*(3.0./5.0e+1)];
mt46 = [th31_dot.*(t10.*t31.*(3.0./5.0e+1)+t3.*t16.*t25.*(3.0./5.0e+1))+zeta_dot.*(t16.*t25.*(3.0./5.0e+1)+t3.*t10.*t31.*(3.0./5.0e+1))+psi_dot.*t10.*t16.*t18.*(3.0./5.0e+1),t118+t167+t324+t350-t376+t528+t635+t643+t662+t748-t799+t872+t1096+t1156-t1241-t1412-t1584+t31.*t436-psi_dot.*t10.*t31.*(3.0./5.0e+2)+t25.*t31.*th31_dot.*(2.1e+1./1.0e+3)-phi_dot.*t10.*t47.*t73.*(3.0./5.0e+2)-psi_dot.*t3.*t10.*t16.*(3.0./2.5e+2)-t3.*t10.*t16.*th31_dot.*(2.1e+1./1.0e+3)+t10.*t16.*t18.*th31_dot.*(3.0./5.0e+2)+t16.*t18.*t25.*th31_dot.*(3.0./2.5e+2)-t18.*t25.*t31.*zeta_dot.*(3.0./5.0e+2)-phi_dot.*t10.*t25.*t47.*t73.*(4.0./3.75e+2)];
mt47 = [t153-t179-t356+t400+t484+t627+t677+t811+t848+t1072+psi_dot.*t10.*t18.*(3.0./2.5e+2)-psi_dot.*t18.*t66.*(4.0./3.75e+2)+t3.*t10.*th31_dot.*(3.0./5.0e+2)+t3.*t25.*th31_dot.*(3.0./2.5e+2)+t10.*t18.*th31_dot.*(2.1e+1./1.0e+3)-phi_dot.*t10.*t16.*t47.*(2.1e+1./1.0e+3),t130+t150+t171+t250+t302-t436-t688+t727-t25.*th31_dot.*(2.1e+1./1.0e+3)-phi_dot.*t10.*t31.*(3.0./5.0e+2)-phi_dot.*t31.*t81.*(2.0./3.75e+2)-t18.*t54.*zeta_dot.*(2.0./3.75e+2)-phi_dot.*t3.*t16.*t25.*(3.0./5.0e+2),0.0,0.0,0.0,0.0,0.0,0.0,0.0,0.0,0.0,0.0,0.0,0.0,0.0,0.0,0.0,0.0,0.0,0.0,0.0,0.0,0.0,0.0,0.0,0.0];
mt48 = [-psi_dot.*(t11.*t724.*(3.0./5.0e+1)+t26.*t92.*t360.*(3.0./1.0e+2))-zeta_dot.*(t26.*t2148.*(3.0./5.0e+1)+t11.*t16.*t88.*(3.0./5.0e+1))-phi_dot.*(t11.*t723.*(3.0./5.0e+1)+t26.*t2178.*(3.0./5.0e+1))+th32_dot.*(t26.*t360.*(3.0./5.0e+1)+t11.*t2179.*(3.0./5.0e+1)),psi_dot.*(t11.*t359.*(3.0./5.0e+1)+t26.*t92.*t723.*(3.0./1.0e+2))-zeta_dot.*(t26.*t2149.*(3.0./5.0e+1)+t11.*t16.*t90.*(3.0./5.0e+1))-phi_dot.*(t11.*t360.*(3.0./5.0e+1)-t26.*t2179.*(3.0./5.0e+1))-th32_dot.*(t26.*t723.*(3.0./5.0e+1)-t11.*t2178.*(3.0./5.0e+1))];
mt49 = [-th32_dot.*(t11.*t1645.*(3.0./5.0e+1)-t3.*t16.*t26.*(3.0./5.0e+1))-t16.*t26.*zeta_dot.*(3.0./1.0e+2)+psi_dot.*t11.*t16.*t18.*(3.0./5.0e+1)+t3.*t11.*t31.*zeta_dot.*(3.0./5.0e+1)-psi_dot.*t3.*t16.*t26.*t92.*(3.0./1.0e+2)+t18.*t26.*t31.*t92.*zeta_dot.*(3.0./1.0e+2),et132+et133];
mt50 = [-t180-t282+t401+t485+t496+t628+t678-t716+t812-t847+t913+t939+t989+t1073+t1142-t1397-t1432-t1466+t1540+t1603-t1633+t1735-t1787+t1803-t1820+t1889+t1966+psi_dot.*t11.*t18.*2.55e-2-t3.*t11.*th32_dot.*(3.0./1.0e+3)+t3.*t26.*th32_dot.*2.55e-2-t11.*t18.*th32_dot.*1.05e-2-phi_dot.*t11.*t16.*t47.*(2.1e+1./1.0e+3)-psi_dot.*t3.*t26.*t92.*1.275e-2-t11.*t18.*t92.*th32_dot.*1.05e-2-t26.*t47.*t92.*zeta_dot.*1.05e-2-phi_dot.*t3.*t16.*t18.*t26.*t92.*1.05e-2];
mt51 = [t131+t160+t185-t278+t298-t320-t365+t442+t450+t542+t576+t704+t929-t1440-t1496-t1736-t1795-t26.*th32_dot.*(2.1e+1./1.0e+3)-phi_dot.*t11.*t31.*(3.0./5.0e+2)-t11.*t92.*th32_dot.*(3.0./1.0e+3)+t26.*t92.*th32_dot.*4.5e-3-phi_dot.*t3.*t16.*t67.*(2.0./3.75e+2)-phi_dot.*t26.*t31.*t92.*1.05e-2,0.0,0.0,0.0,0.0,0.0,0.0,0.0,0.0,0.0,0.0,0.0,0.0,0.0,0.0,0.0,0.0,0.0,0.0,0.0,0.0,0.0,0.0,0.0,0.0];
mt52 = [-psi_dot.*(t12.*t724.*(3.0./5.0e+1)-t27.*t92.*t360.*(3.0./1.0e+2))-zeta_dot.*(t27.*t2175.*(3.0./5.0e+1)+t12.*t16.*t88.*(3.0./5.0e+1))-phi_dot.*(t12.*t723.*(3.0./5.0e+1)+t27.*t2177.*(3.0./5.0e+1))+th33_dot.*(t27.*t360.*(3.0./5.0e+1)+t12.*t2180.*(3.0./5.0e+1)),psi_dot.*(t12.*t359.*(3.0./5.0e+1)-t27.*t92.*t723.*(3.0./1.0e+2))-zeta_dot.*(t27.*t2176.*(3.0./5.0e+1)+t12.*t16.*t90.*(3.0./5.0e+1))-phi_dot.*(t12.*t360.*(3.0./5.0e+1)-t27.*t2180.*(3.0./5.0e+1))-th33_dot.*(t27.*t723.*(3.0./5.0e+1)-t12.*t2177.*(3.0./5.0e+1))];
mt53 = [-th33_dot.*(t12.*t1840.*(3.0./5.0e+1)-t3.*t16.*t27.*(3.0./5.0e+1))-t16.*t27.*zeta_dot.*(3.0./1.0e+2)+psi_dot.*t12.*t16.*t18.*(3.0./5.0e+1)+t3.*t12.*t31.*zeta_dot.*(3.0./5.0e+1)+psi_dot.*t3.*t16.*t27.*t92.*(3.0./1.0e+2)-t18.*t27.*t31.*t92.*zeta_dot.*(3.0./1.0e+2),et134+et135];
mt54 = [-t181-t283+t402+t486+t498+t629+t679-t718+t813-t849+t914-t940+t1074+t1143+t1174+t1392+t1398+t1433+t1467+t1634+t1696+t1788-t1804+t1821-t1967+t2031+psi_dot.*t12.*t18.*2.55e-2-t3.*t12.*th33_dot.*(3.0./1.0e+3)+t3.*t27.*th33_dot.*2.55e-2-t12.*t18.*th33_dot.*1.05e-2-phi_dot.*t12.*t16.*t47.*(2.1e+1./1.0e+3)+psi_dot.*t3.*t27.*t92.*1.275e-2+t12.*t18.*t92.*th33_dot.*1.05e-2-phi_dot.*t12.*t16.*t47.*t92.*4.5e-3-t3.*t18.*t27.*t92.*zeta_dot.*(3.0./1.0e+3)-(phi_dot.*t3.*t12.*t27.*t31.*t92)./3.75e+2];
mt55 = [t132+t160+t185-t279+t299-t321-t366+t443+t451+t543+t578+t706-t930+t1321+t1441+t1497+t1738+t1796-t27.*th33_dot.*(2.1e+1./1.0e+3)-phi_dot.*t12.*t31.*(3.0./5.0e+2)+t12.*t92.*th33_dot.*(3.0./1.0e+3)-t27.*t92.*th33_dot.*4.5e-3-phi_dot.*t3.*t16.*t68.*(2.0./3.75e+2),0.0,0.0,0.0,0.0,0.0,0.0,0.0,0.0,0.0,0.0,0.0,0.0,0.0,0.0,0.0,0.0,0.0,0.0,0.0,0.0,0.0,0.0,0.0,0.0,0.0,0.0,0.0,0.0,0.0,0.0,0.0,0.0,0.0,0.0,0.0,0.0,0.0,0.0,0.0,0.0,0.0,0.0,0.0,0.0,0.0,0.0,0.0,0.0,0.0,0.0,0.0,0.0,0.0,0.0,0.0,0.0,0.0,0.0,0.0,0.0,0.0,0.0,0.0,0.0,0.0,0.0,0.0,0.0,0.0,0.0,0.0,0.0,0.0,0.0,0.0,0.0,0.0,0.0,0.0,0.0,0.0,0.0,0.0,0.0,0.0,0.0,0.0,0.0,0.0,0.0,0.0,0.0,0.0,0.0,0.0,0.0,0.0,0.0,0.0,0.0,0.0,0.0,0.0,0.0,0.0,0.0,0.0,0.0,0.0,0.0,0.0,0.0,0.0,0.0];
mt56 = [-phi_dot.*(t13.*t723.*(3.0./5.0e+1)-t16.*t17.*t28.*(3.0./5.0e+1))+th41_dot.*(t28.*t360.*(3.0./5.0e+1)-t2.*t13.*t16.*(3.0./5.0e+1))+zeta_dot.*((t2.*t993)./1.0e+2+t2.*t28.*t31.*(3.0./1.0e+2)-t13.*t16.*t88.*(3.0./1.0e+2))-psi_dot.*t13.*t724.*(3.0./5.0e+1),-phi_dot.*(t13.*t360.*(3.0./5.0e+1)+t2.*t16.*t28.*(3.0./5.0e+1))-th41_dot.*(t28.*t723.*(3.0./5.0e+1)+t13.*t16.*t17.*(3.0./5.0e+1))+zeta_dot.*((t17.*t993)./1.0e+2+t17.*t28.*t31.*(3.0./1.0e+2)-t13.*t16.*t90.*(3.0./1.0e+2))+psi_dot.*t13.*t359.*(3.0./5.0e+1)];
mt57 = [th41_dot.*(t13.*t31.*(3.0./5.0e+1)+t3.*t16.*t28.*(3.0./5.0e+1))+zeta_dot.*(t16.*t28.*(3.0./5.0e+1)+t3.*t13.*t31.*(3.0./5.0e+1))+psi_dot.*t13.*t16.*t18.*(3.0./5.0e+1),t121+t168+t324+t350-t379+t529+t636+t646+t664+t751-t802+t875+t1099+t1244-t1413+t1587-psi_dot.*t13.*t31.*(3.0./5.0e+2)-t28.*t31.*th41_dot.*(2.1e+1./1.0e+3)-phi_dot.*t13.*t47.*t73.*(3.0./5.0e+2)-psi_dot.*t3.*t13.*t16.*(3.0./2.5e+2)+t3.*t13.*t16.*th41_dot.*(2.1e+1./1.0e+3)+t13.*t16.*t18.*th41_dot.*(3.0./5.0e+2)+t16.*t18.*t28.*th41_dot.*(3.0./2.5e+2)-t3.*t28.*t31.*zeta_dot.*(2.1e+1./1.0e+3)-t18.*t28.*t31.*zeta_dot.*(3.0./5.0e+2)-phi_dot.*t16.*t18.*t28.*t31.*(2.1e+1./1.0e+3)-phi_dot.*t13.*t28.*t47.*t73.*(4.0./3.75e+2)];
mt58 = [t154-t182-t358-t403+t487+t630-t680+t814+t851+t1075+t1212+psi_dot.*t13.*t18.*(3.0./2.5e+2)-psi_dot.*t18.*t69.*(4.0./3.75e+2)+t3.*t13.*th41_dot.*(3.0./5.0e+2)+t3.*t28.*th41_dot.*(3.0./2.5e+2)-t13.*t18.*th41_dot.*(2.1e+1./1.0e+3),t133+t150+t172+t251+t302+t437+t690+t728+t28.*th41_dot.*(2.1e+1./1.0e+3)-phi_dot.*t13.*t31.*(3.0./5.0e+2)-phi_dot.*t31.*t84.*(2.0./3.75e+2)-t18.*t57.*zeta_dot.*(2.0./3.75e+2)-phi_dot.*t3.*t16.*t28.*(3.0./5.0e+2),0.0,0.0,0.0,0.0,0.0,0.0,0.0,0.0,0.0,0.0,0.0,0.0,0.0,0.0,0.0,0.0,0.0,0.0,0.0,0.0,0.0,0.0,0.0,0.0];
mt59 = [-psi_dot.*(t14.*t724.*(3.0./5.0e+1)+t29.*t92.*t360.*(3.0./1.0e+2))-zeta_dot.*(t29.*t2148.*(3.0./5.0e+1)+t14.*t16.*t88.*(3.0./5.0e+1))-phi_dot.*(t14.*t723.*(3.0./5.0e+1)+t29.*t2178.*(3.0./5.0e+1))+th42_dot.*(t29.*t360.*(3.0./5.0e+1)+t14.*t2179.*(3.0./5.0e+1)),psi_dot.*(t14.*t359.*(3.0./5.0e+1)+t29.*t92.*t723.*(3.0./1.0e+2))-zeta_dot.*(t29.*t2149.*(3.0./5.0e+1)+t14.*t16.*t90.*(3.0./5.0e+1))-phi_dot.*(t14.*t360.*(3.0./5.0e+1)-t29.*t2179.*(3.0./5.0e+1))-th42_dot.*(t29.*t723.*(3.0./5.0e+1)-t14.*t2178.*(3.0./5.0e+1))];
mt60 = [-th42_dot.*(t14.*t1645.*(3.0./5.0e+1)-t3.*t16.*t29.*(3.0./5.0e+1))-t16.*t29.*zeta_dot.*(3.0./1.0e+2)+psi_dot.*t14.*t16.*t18.*(3.0./5.0e+1)+t3.*t14.*t31.*zeta_dot.*(3.0./5.0e+1)-psi_dot.*t3.*t16.*t29.*t92.*(3.0./1.0e+2)+t18.*t29.*t31.*t92.*zeta_dot.*(3.0./1.0e+2),et136+et137];
mt61 = [-t183-t284-t404+t488+t499+t631-t681-t720+t815-t850+t915-t941+t989+t1076+t1144+t1213-t1399-t1434-t1470+t1540+t1605-t1635+t1697+t1739-t1789+t1805-t1822+t1891+t1968+t2032+psi_dot.*t14.*t18.*2.55e-2-t3.*t14.*th42_dot.*(3.0./1.0e+3)+t3.*t29.*th42_dot.*2.55e-2+t14.*t18.*th42_dot.*1.05e-2-psi_dot.*t3.*t29.*t92.*1.275e-2-t14.*t18.*t92.*th42_dot.*1.05e-2];
mt62 = [t134+t160+t185-t280+t300-t322-t367-t444+t452+t544+t580-t712-t931+t1322-t1442-t1498-t1740-t1799+t29.*th42_dot.*(2.1e+1./1.0e+3)-phi_dot.*t14.*t31.*(3.0./5.0e+2)-t14.*t92.*th42_dot.*(3.0./1.0e+3)+t29.*t92.*th42_dot.*4.5e-3-phi_dot.*t3.*t16.*t70.*(2.0./3.75e+2),0.0,0.0,0.0,0.0,0.0,0.0,0.0,0.0,0.0,0.0,0.0,0.0,0.0,0.0,0.0,0.0,0.0,0.0,0.0,0.0,0.0,0.0,0.0,0.0];
mt63 = [-psi_dot.*(t15.*t724.*(3.0./5.0e+1)-t30.*t92.*t360.*(3.0./1.0e+2))-zeta_dot.*(t30.*t2175.*(3.0./5.0e+1)+t15.*t16.*t88.*(3.0./5.0e+1))-phi_dot.*(t15.*t723.*(3.0./5.0e+1)+t30.*t2177.*(3.0./5.0e+1))+th43_dot.*(t30.*t360.*(3.0./5.0e+1)+t15.*t2180.*(3.0./5.0e+1)),psi_dot.*(t15.*t359.*(3.0./5.0e+1)-t30.*t92.*t723.*(3.0./1.0e+2))-zeta_dot.*(t30.*t2176.*(3.0./5.0e+1)+t15.*t16.*t90.*(3.0./5.0e+1))-phi_dot.*(t15.*t360.*(3.0./5.0e+1)-t30.*t2180.*(3.0./5.0e+1))-th43_dot.*(t30.*t723.*(3.0./5.0e+1)-t15.*t2177.*(3.0./5.0e+1))];
mt64 = [-th43_dot.*(t15.*t1840.*(3.0./5.0e+1)-t3.*t16.*t30.*(3.0./5.0e+1))-t16.*t30.*zeta_dot.*(3.0./1.0e+2)+psi_dot.*t15.*t16.*t18.*(3.0./5.0e+1)+t3.*t15.*t31.*zeta_dot.*(3.0./5.0e+1)+psi_dot.*t3.*t16.*t30.*t92.*(3.0./1.0e+2)-t18.*t30.*t31.*t92.*zeta_dot.*(3.0./1.0e+2),et138+et139];
mt65 = [-t184-t285-t405+t489+t501+t632-t682-t722+t816-t852+t916+t942+t1077+t1145+t1174+t1214+t1392+t1400+t1435+t1471+t1636+t1790-t1806+t1823-t1969+psi_dot.*t15.*t18.*2.55e-2-t3.*t15.*th43_dot.*(3.0./1.0e+3)+t3.*t30.*th43_dot.*2.55e-2+t15.*t18.*th43_dot.*1.05e-2+psi_dot.*t3.*t30.*t92.*1.275e-2+t15.*t18.*t92.*th43_dot.*1.05e-2-t30.*t47.*t92.*zeta_dot.*1.05e-2-phi_dot.*t15.*t16.*t47.*t92.*4.5e-3-t3.*t18.*t30.*t92.*zeta_dot.*(3.0./1.0e+3)-phi_dot.*t3.*t16.*t18.*t30.*t92.*1.05e-2-(phi_dot.*t3.*t15.*t30.*t31.*t92)./3.75e+2];
mt66 = [t135+t160+t185-t281+t301-t323-t368-t445+t453+t545+t582-t714+t932+t1443+t1499+t1742+t1800+t30.*th43_dot.*(2.1e+1./1.0e+3)-phi_dot.*t15.*t31.*(3.0./5.0e+2)+t15.*t92.*th43_dot.*(3.0./1.0e+3)-t30.*t92.*th43_dot.*4.5e-3-phi_dot.*t3.*t16.*t71.*(2.0./3.75e+2)-phi_dot.*t30.*t31.*t92.*1.05e-2,0.0,0.0,0.0,0.0,0.0,0.0,0.0,0.0,0.0,0.0,0.0,0.0,0.0,0.0,0.0,0.0,0.0,0.0,0.0,0.0,0.0,0.0,0.0,0.0,0.0,0.0,0.0,0.0,0.0,0.0,0.0,0.0,0.0,0.0,0.0,0.0,0.0,0.0,0.0,0.0,0.0,0.0,0.0,0.0,0.0,0.0,0.0,0.0,0.0,0.0,0.0,0.0,0.0,0.0,0.0,0.0,0.0,0.0,0.0,0.0,0.0,0.0,0.0,0.0,0.0,0.0,0.0,0.0,0.0,0.0,0.0,0.0,0.0,0.0,0.0,0.0,0.0,0.0,0.0,0.0,0.0,0.0,0.0,0.0,0.0,0.0,0.0,0.0,0.0,0.0,0.0,0.0,0.0,0.0,0.0,0.0,0.0,0.0,0.0,0.0,0.0];
mt67 = [0.0,0.0,0.0,0.0,0.0,0.0,0.0,0.0,0.0,0.0,0.0,0.0,0.0];
C = reshape([mt1,mt2,mt3,mt4,mt5,mt6,mt7,mt8,mt9,mt10,mt11,mt12,mt13,mt14,mt15,mt16,mt17,mt18,mt19,mt20,mt21,mt22,mt23,mt24,mt25,mt26,mt27,mt28,mt29,mt30,mt31,mt32,mt33,mt34,mt35,mt36,mt37,mt38,mt39,mt40,mt41,mt42,mt43,mt44,mt45,mt46,mt47,mt48,mt49,mt50,mt51,mt52,mt53,mt54,mt55,mt56,mt57,mt58,mt59,mt60,mt61,mt62,mt63,mt64,mt65,mt66,mt67],30,30);
end
